simulink model "model"  (R2016a)
(part 9 of 10)

  _CN_101346507_220000_CN_101346508_220000/RConn1 -- T_101346508_220000_Ital_Novi/LConn1 -- Vignole_Ilva_CN_101346508_220000_CN_100952845_220000/RConn1
  _CN_101346507_220000_CN_101346508_220000/RConn2 -- T_101346508_220000_Ital_Novi/LConn2 -- Vignole_Ilva_CN_101346508_220000_CN_100952845_220000/RConn2
  _CN_101346507_220000_CN_101346508_220000/RConn3 -- T_101346508_220000_Ital_Novi/LConn3 -- Vignole_Ilva_CN_101346508_220000_CN_100952845_220000/RConn3 -- bus206/LConn1
  T_95466193_220000_/LConn1 -- Roma_Sud_Cinecittà_CN_95466193_220000_CN_76705565_220000/LConn1
  T_95466193_220000_/LConn2 -- Roma_Sud_Cinecittà_CN_95466193_220000_CN_76705565_220000/LConn2
  Roma_Sud_Cinecittà_CN_95466193_220000_CN_76705565_220000/LConn3 -- T_95466193_220000_/LConn3 -- bus207/LConn1
  Roma_Sud_Cinecittà_CN_95466193_220000_CN_76705565_220000/RConn1 -- T_76705565_380000;220000;150000_Roma_Sud/RConn1 -- Roma_Sud_San_Paolo_CN_76705565_220000_CN_95466377_220000/LConn1
  Roma_Sud_Cinecittà_CN_95466193_220000_CN_76705565_220000/RConn2 -- T_76705565_380000;220000;150000_Roma_Sud/RConn2 -- Roma_Sud_San_Paolo_CN_76705565_220000_CN_95466377_220000/LConn2
  Roma_Sud_Cinecittà_CN_95466193_220000_CN_76705565_220000/RConn3 -- T_76705565_380000;220000;150000_Roma_Sud/RConn3 -- Roma_Sud_San_Paolo_CN_76705565_220000_CN_95466377_220000/LConn3 -- bus208/LConn1
  _CN_375916035_220000_CN_56984450_220000/RConn1 -- T_375916035_220000_Cattolica_Eraclea_centrale/LConn1 -- _CN_375916035_220000_CN_53635045_220000/RConn1 -- _CN_375916035_220000_CN_375907988_220000/LConn1
  _CN_375916035_220000_CN_56984450_220000/RConn2 -- T_375916035_220000_Cattolica_Eraclea_centrale/LConn2 -- _CN_375916035_220000_CN_53635045_220000/RConn2 -- _CN_375916035_220000_CN_375907988_220000/LConn2
  _CN_375916035_220000_CN_56984450_220000/RConn3 -- T_375916035_220000_Cattolica_Eraclea_centrale/LConn3 -- _CN_375916035_220000_CN_53635045_220000/RConn3 -- _CN_375916035_220000_CN_375907988_220000/LConn3 -- bus209/LConn1
  T_375907988_220000_Sambuca/LConn1 -- _CN_375916035_220000_CN_375907988_220000/RConn1
  T_375907988_220000_Sambuca/LConn2 -- _CN_375916035_220000_CN_375907988_220000/RConn2
  _CN_375916035_220000_CN_375907988_220000/RConn3 -- T_375907988_220000_Sambuca/LConn3 -- bus210/LConn1
  Patria_Pozzuoli_CN_114661587_220000_CN_132726160_220000/RConn1 -- T_132726160_220000_Pozzuoli/LConn1 -- Astroni_Pozzuoli_CN_132726160_220000_CN_132725149_220000/RConn1
  Patria_Pozzuoli_CN_114661587_220000_CN_132726160_220000/RConn2 -- T_132726160_220000_Pozzuoli/LConn2 -- Astroni_Pozzuoli_CN_132726160_220000_CN_132725149_220000/RConn2
  Patria_Pozzuoli_CN_114661587_220000_CN_132726160_220000/RConn3 -- T_132726160_220000_Pozzuoli/LConn3 -- Astroni_Pozzuoli_CN_132726160_220000_CN_132725149_220000/RConn3 -- bus211/LConn1
  T_377832777_220000_Tirano/LConn1 -- Cesano_Maderno_Tirano_CN_74359510_220000_CN_377832777_220000/RConn1
  T_377832777_220000_Tirano/LConn2 -- Cesano_Maderno_Tirano_CN_74359510_220000_CN_377832777_220000/RConn2
  Cesano_Maderno_Tirano_CN_74359510_220000_CN_377832777_220000/RConn3 -- T_377832777_220000_Tirano/LConn3 -- bus212/LConn1
  Cesano_Maderno_Tirano_CN_74359510_220000_CN_98787157_220000/RConn1 -- T_98787157_220000_Glorenza/LConn1 -- _CN_98787157_220000_CN96653153/LConn1
  Cesano_Maderno_Tirano_CN_74359510_220000_CN_98787157_220000/RConn2 -- T_98787157_220000_Glorenza/LConn2 -- _CN_98787157_220000_CN96653153/LConn2
  Cesano_Maderno_Tirano_CN_74359510_220000_CN_98787157_220000/RConn3 -- T_98787157_220000_Glorenza/LConn3 -- _CN_98787157_220000_CN96653153/LConn3 -- bus213/LConn1
  T_377588184_220000_Caivano/LConn1 -- Fratta_Maddaloni_CN_132702940_220000_CN_377588184_220000/RConn1
  T_377588184_220000_Caivano/LConn2 -- Fratta_Maddaloni_CN_132702940_220000_CN_377588184_220000/RConn2
  Fratta_Maddaloni_CN_132702940_220000_CN_377588184_220000/RConn3 -- T_377588184_220000_Caivano/LConn3 -- bus214/LConn1
  T_132719324_220000_Air_Liquide/LConn1 -- Maddaloni_Air_Liquide_CN_132719324_220000_CN_132717802_220000/RConn1
  T_132719324_220000_Air_Liquide/LConn2 -- Maddaloni_Air_Liquide_CN_132719324_220000_CN_132717802_220000/RConn2
  Maddaloni_Air_Liquide_CN_132719324_220000_CN_132717802_220000/RConn3 -- T_132719324_220000_Air_Liquide/LConn3 -- bus215/LConn1
  T_84696559_380000_Santa_Sofia/RConn4 -- Maddaloni_Santa_Sofia_CN_132717802_220000_CN_84696559_220000/RConn1
  T_84696559_380000_Santa_Sofia/RConn5 -- Maddaloni_Santa_Sofia_CN_132717802_220000_CN_84696559_220000/RConn2
  Maddaloni_Santa_Sofia_CN_132717802_220000_CN_84696559_220000/RConn3 -- T_84696559_380000_Santa_Sofia/RConn6 -- bus216/LConn1
  T_162960205_380000_Tavazzano_Centrale/RConn4 -- _CN_116916459_220000_CN_162960205_220000/RConn1
  T_162960205_380000_Tavazzano_Centrale/RConn5 -- _CN_116916459_220000_CN_162960205_220000/RConn2
  _CN_116916459_220000_CN_162960205_220000/RConn3 -- T_162960205_380000_Tavazzano_Centrale/RConn6 -- bus217/LConn1
  T_214294769_220000_Moline/LConn1 -- _CN_214294769_220000_CN_103549584_220000/RConn1
  T_214294769_220000_Moline/LConn2 -- _CN_214294769_220000_CN_103549584_220000/RConn2
  _CN_214294769_220000_CN_103549584_220000/RConn3 -- T_214294769_220000_Moline/LConn3 -- bus218/LConn1
  T_281837810_220000_Cedegolo_Sud/LConn1 -- Taio_Cedegolo_CN_281837810_220000_CN96654904/RConn1
  T_281837810_220000_Cedegolo_Sud/LConn2 -- Taio_Cedegolo_CN_281837810_220000_CN96654904/RConn2
  Taio_Cedegolo_CN_281837810_220000_CN96654904/RConn3 -- T_281837810_220000_Cedegolo_Sud/LConn3 -- bus219/LConn1
  T_181125039_220000_Enipower_Ferrara/LConn1 -- Bussolengo_Ferrara_CN_111020792_220000_CN_181125039_220000/RConn1
  T_181125039_220000_Enipower_Ferrara/LConn2 -- Bussolengo_Ferrara_CN_111020792_220000_CN_181125039_220000/RConn2
  Bussolengo_Ferrara_CN_111020792_220000_CN_181125039_220000/RConn3 -- T_181125039_220000_Enipower_Ferrara/LConn3 -- bus220/LConn1
  T_82078641_380000_Ostiglia/RConn4 -- Mincio_Colunga_CN_111020792_220000_CN_82078641_220000/RConn1
  T_82078641_380000_Ostiglia/RConn5 -- Mincio_Colunga_CN_111020792_220000_CN_82078641_220000/RConn2
  Mincio_Colunga_CN_111020792_220000_CN_82078641_220000/RConn3 -- T_82078641_380000_Ostiglia/RConn6 -- bus221/LConn1
  T_162066058_220000_Verona_Borgomilano/LConn1 -- _CN_111020792_220000_CN_162066058_220000/RConn1
  T_162066058_220000_Verona_Borgomilano/LConn2 -- _CN_111020792_220000_CN_162066058_220000/RConn2
  _CN_111020792_220000_CN_162066058_220000/RConn3 -- T_162066058_220000_Verona_Borgomilano/LConn3 -- bus222/LConn1
  T_289178949_220000_Riva_Acciaio/LConn1 -- _CN_111020792_220000_CN_289178949_220000/RConn1
  T_289178949_220000_Riva_Acciaio/LConn2 -- _CN_111020792_220000_CN_289178949_220000/RConn2
  _CN_111020792_220000_CN_289178949_220000/RConn3 -- T_289178949_220000_Riva_Acciaio/LConn3 -- bus223/LConn1
  T_103725446_220000_Sondel_Settimo_Torinese/LConn1 -- Stura_Sondel_CN_103725268_220000_CN_103725446_220000/RConn1
  T_103725446_220000_Sondel_Settimo_Torinese/LConn2 -- Stura_Sondel_CN_103725268_220000_CN_103725446_220000/RConn2
  Stura_Sondel_CN_103725268_220000_CN_103725446_220000/RConn3 -- T_103725446_220000_Sondel_Settimo_Torinese/LConn3 -- bus224/LConn1
  T_82767145_380000_Tirreno_Power_Torrevaldaliga/RConn4 -- Torrevaldaliga_Sud_Santa_Lucia_CN_82762493_220000_CN_82767145_220000/RConn1
  T_82767145_380000_Tirreno_Power_Torrevaldaliga/RConn5 -- Torrevaldaliga_Sud_Santa_Lucia_CN_82762493_220000_CN_82767145_220000/RConn2
  Torrevaldaliga_Sud_Santa_Lucia_CN_82762493_220000_CN_82767145_220000/RConn3 -- T_82767145_380000_Tirreno_Power_Torrevaldaliga/RConn6 -- bus225/LConn1
  T_194186027_220000_Duferdofin/LConn1 -- Sorgente___Duferdofin_CN_194186027_220000_CN_110138220_220000/RConn1
  T_194186027_220000_Duferdofin/LConn2 -- Sorgente___Duferdofin_CN_194186027_220000_CN_110138220_220000/RConn2
  Sorgente___Duferdofin_CN_194186027_220000_CN_110138220_220000/RConn3 -- T_194186027_220000_Duferdofin/LConn3 -- bus226/LConn1
  T_338948868_220000_Termini_Centrale_gruppi_6/LConn1 -- _CN_338948868_220000_CN53456167/LConn1
  T_338948868_220000_Termini_Centrale_gruppi_6/LConn2 -- _CN_338948868_220000_CN53456167/LConn2
  _CN_338948868_220000_CN53456167/LConn3 -- T_338948868_220000_Termini_Centrale_gruppi_6/LConn3 -- bus227/LConn1
  _CN_338948868_220000_CN53456167/RConn1 -- "G_53456167_Centrale_termoelettrica_\"Ettore_Maiorana\""/RConn1 -- _CN_57736553_220000_CN53456167/RConn1
  _CN_338948868_220000_CN53456167/RConn2 -- "G_53456167_Centrale_termoelettrica_\"Ettore_Maiorana\""/RConn2 -- _CN_57736553_220000_CN53456167/RConn2
  _CN_338948868_220000_CN53456167/RConn3 -- "G_53456167_Centrale_termoelettrica_\"Ettore_Maiorana\""/RConn3 -- _CN_57736553_220000_CN53456167/RConn3 -- bus228/LConn1
  T_145665797_220000_Brindisi_Nord_220/LConn1 -- Brindisi_Brindisi_Nord_CN_145665797_220000_CN402304796/LConn1
  T_145665797_220000_Brindisi_Nord_220/LConn2 -- Brindisi_Brindisi_Nord_CN_145665797_220000_CN402304796/LConn2
  Brindisi_Brindisi_Nord_CN_145665797_220000_CN402304796/LConn3 -- T_145665797_220000_Brindisi_Nord_220/LConn3 -- bus229/LConn1
  Brindisi_Brindisi_Nord_CN_145665797_220000_CN402304796/RConn1 -- G_402304796_Centrale_termoelettrica_di_Brindisi/RConn1 -- Brindisi_Brindisi_Nord_CN_60919237_220000_CN402304796/LConn1
  Brindisi_Brindisi_Nord_CN_145665797_220000_CN402304796/RConn2 -- G_402304796_Centrale_termoelettrica_di_Brindisi/RConn2 -- Brindisi_Brindisi_Nord_CN_60919237_220000_CN402304796/LConn2
  Brindisi_Brindisi_Nord_CN_145665797_220000_CN402304796/RConn3 -- G_402304796_Centrale_termoelettrica_di_Brindisi/RConn3 -- Brindisi_Brindisi_Nord_CN_60919237_220000_CN402304796/LConn3 -- bus230/LConn1
  T_103653591_220000_Vado_Stazione/LConn1 -- Savona_Vado_Ligure_CN_103653591_220000_CN_296141722_220000/RConn1
  T_103653591_220000_Vado_Stazione/LConn2 -- Savona_Vado_Ligure_CN_103653591_220000_CN_296141722_220000/RConn2
  Savona_Vado_Ligure_CN_103653591_220000_CN_296141722_220000/RConn3 -- T_103653591_220000_Vado_Stazione/LConn3 -- bus231/LConn1
  T_100407576_380000_Fusina_Termica_sezione_1_220/RConn1 -- Dolo___Fusina_CN_100407576_220000_CN_59153311_220000/RConn1
  T_100407576_380000_Fusina_Termica_sezione_1_220/RConn2 -- Dolo___Fusina_CN_100407576_220000_CN_59153311_220000/RConn2
  Dolo___Fusina_CN_100407576_220000_CN_59153311_220000/RConn3 -- T_100407576_380000_Fusina_Termica_sezione_1_220/RConn3 -- bus232/LConn1
  T_95466377_220000_/LConn1 -- Roma_Sud_San_Paolo_CN_76705565_220000_CN_95466377_220000/RConn1
  T_95466377_220000_/LConn2 -- Roma_Sud_San_Paolo_CN_76705565_220000_CN_95466377_220000/RConn2
  Roma_Sud_San_Paolo_CN_76705565_220000_CN_95466377_220000/RConn3 -- T_95466377_220000_/LConn3 -- bus233/LConn1
  Villa___Rosone_CN_66872608_220000_CN_102185356_220000/RConn1 -- T_102185356_220000_Villa/LConn1 -- Villeneuve_Villa_CN_102185356_220000_CN_102185362_220000/RConn1
  Villa___Rosone_CN_66872608_220000_CN_102185356_220000/RConn2 -- T_102185356_220000_Villa/LConn2 -- Villeneuve_Villa_CN_102185356_220000_CN_102185362_220000/RConn2
  Villa___Rosone_CN_66872608_220000_CN_102185356_220000/RConn3 -- T_102185356_220000_Villa/LConn3 -- Villeneuve_Villa_CN_102185356_220000_CN_102185362_220000/RConn3 -- bus234/LConn1
  T_162828577_380000_Turbigo/RConn4 -- Biella_Est___Turbigo_CN_162828577_220000_CN_82651599_220000/RConn1
  T_162828577_380000_Turbigo/RConn5 -- Biella_Est___Turbigo_CN_162828577_220000_CN_82651599_220000/RConn2
  Biella_Est___Turbigo_CN_162828577_220000_CN_82651599_220000/RConn3 -- T_162828577_380000_Turbigo/RConn6 -- bus235/LConn1
  T_136708548_220000_Certosa/LConn1 -- _CN_62326314_220000_CN_136708548_220000/RConn1
  T_136708548_220000_Certosa/LConn2 -- _CN_62326314_220000_CN_136708548_220000/RConn2
  _CN_62326314_220000_CN_136708548_220000/RConn3 -- T_136708548_220000_Certosa/LConn3 -- bus236/LConn1
  T_118987056_380000_Selargius/RConn4 -- Selargius_Villasor_CN_118987056_220000_CN_144005861_220000/RConn1
  T_118987056_380000_Selargius/RConn5 -- Selargius_Villasor_CN_118987056_220000_CN_144005861_220000/RConn2
  Selargius_Villasor_CN_118987056_220000_CN_144005861_220000/RConn3 -- T_118987056_380000_Selargius/RConn6 -- bus237/LConn1
  Colli_Aminei_Secondigliano_CN_377444657_220000_CN_376502663_220000/RConn1 -- T_377444657_220000_Secondigliano/LConn1 -- Fratta_Secondigliano_CN_377444657_220000_CN_377444648_220000/RConn1
  Colli_Aminei_Secondigliano_CN_377444657_220000_CN_376502663_220000/RConn2 -- T_377444657_220000_Secondigliano/LConn2 -- Fratta_Secondigliano_CN_377444657_220000_CN_377444648_220000/RConn2
  Colli_Aminei_Secondigliano_CN_377444657_220000_CN_376502663_220000/RConn3 -- T_377444657_220000_Secondigliano/LConn3 -- Fratta_Secondigliano_CN_377444657_220000_CN_377444648_220000/RConn3 -- bus238/LConn1
  _CN_172705586_220000_CN_57736541_220000/LConn1 -- T_172705586__Bellolampo/LConn1 -- _CN_172705586_220000_CN_57736553_220000/RConn1
  _CN_172705586_220000_CN_57736541_220000/LConn2 -- T_172705586__Bellolampo/LConn2 -- _CN_172705586_220000_CN_57736553_220000/RConn2
  _CN_172705586_220000_CN_57736541_220000/LConn3 -- T_172705586__Bellolampo/LConn3 -- _CN_172705586_220000_CN_57736553_220000/RConn3 -- bus239/LConn1
  _CN_172705586_220000_CN_57736541_220000/RConn1 -- T_57736541__Partinico/LConn1 -- _CN_57736541_220000_CN_57403755_220000/LConn1 -- _CN_57736541_220000_CN_53635045_220000/RConn1
  _CN_172705586_220000_CN_57736541_220000/RConn2 -- T_57736541__Partinico/LConn2 -- _CN_57736541_220000_CN_57403755_220000/LConn2 -- _CN_57736541_220000_CN_53635045_220000/RConn2
  _CN_172705586_220000_CN_57736541_220000/RConn3 -- T_57736541__Partinico/LConn3 -- _CN_57736541_220000_CN_57403755_220000/LConn3 -- _CN_57736541_220000_CN_53635045_220000/RConn3 -- bus240/LConn1
  _CN_103007030_220000_CN_103007085_220000/LConn1 -- T_103007030_220000_Chatillon_Centrale/LConn1 -- _CN_103007030_220000_CN_103127417_220000/LConn1 -- _CN_103007030_220000_CN_102185362_220000/RConn1 -- _CN_103007030_220000_CN_105153431_220000/LConn1
  _CN_103007030_220000_CN_103007085_220000/LConn2 -- T_103007030_220000_Chatillon_Centrale/LConn2 -- _CN_103007030_220000_CN_103127417_220000/LConn2 -- _CN_103007030_220000_CN_102185362_220000/RConn2 -- _CN_103007030_220000_CN_105153431_220000/LConn2
  _CN_103007030_220000_CN_103007085_220000/LConn3 -- T_103007030_220000_Chatillon_Centrale/LConn3 -- _CN_103007030_220000_CN_103127417_220000/LConn3 -- _CN_103007030_220000_CN_102185362_220000/RConn3 -- bus241/LConn1 -- _CN_103007030_220000_CN_105153431_220000/LConn3
  T_103007085_220000_Montjovet_centrale/LConn1 -- _CN_103007030_220000_CN_103007085_220000/RConn1
  T_103007085_220000_Montjovet_centrale/LConn2 -- _CN_103007030_220000_CN_103007085_220000/RConn2
  _CN_103007030_220000_CN_103007085_220000/RConn3 -- T_103007085_220000_Montjovet_centrale/LConn3 -- bus242/LConn1
  _CN_103007030_220000_CN_105153431_220000/RConn1 -- T_105153431_380000_Leinì/RConn4 -- _CN_74869121_220000_CN_105153431_220000/RConn1 -- _CN_105153431_220000_CN_332123606_220000/RConn1
  _CN_103007030_220000_CN_105153431_220000/RConn2 -- T_105153431_380000_Leinì/RConn5 -- _CN_74869121_220000_CN_105153431_220000/RConn2 -- _CN_105153431_220000_CN_332123606_220000/RConn2
  _CN_103007030_220000_CN_105153431_220000/RConn3 -- T_105153431_380000_Leinì/RConn6 -- _CN_74869121_220000_CN_105153431_220000/RConn3 -- _CN_105153431_220000_CN_332123606_220000/RConn3 -- bus243/LConn1
  T_103127417_220000_Valpelline_G2/LConn1 -- _CN_103007030_220000_CN_103127417_220000/RConn1
  T_103127417_220000_Valpelline_G2/LConn2 -- _CN_103007030_220000_CN_103127417_220000/RConn2
  _CN_103007030_220000_CN_103127417_220000/RConn3 -- T_103127417_220000_Valpelline_G2/LConn3 -- bus244/LConn1
  T_189137043_220000_Gargnano/LConn1 -- Gargnano_Nave_CN_189137043_220000_CN_147466201_220000/RConn1
  T_189137043_220000_Gargnano/LConn2 -- Gargnano_Nave_CN_189137043_220000_CN_147466201_220000/RConn2
  Gargnano_Nave_CN_189137043_220000_CN_147466201_220000/RConn3 -- T_189137043_220000_Gargnano/LConn3 -- bus245/LConn1
  G_139974542_Centrale_elettrica_Taloro/RConn1 -- Ottana_Taloro_1_CN_144006711_220000_CN139974542/RConn1
  G_139974542_Centrale_elettrica_Taloro/RConn2 -- Ottana_Taloro_1_CN_144006711_220000_CN139974542/RConn2
  Ottana_Taloro_1_CN_144006711_220000_CN139974542/RConn3 -- G_139974542_Centrale_elettrica_Taloro/RConn3 -- bus246/LConn1
  T_320030656_220000_Tecnoparco/LConn1 -- Pisticci_Tecnoparco_CN_104321356_220000_CN_320030656_220000/RConn1
  T_320030656_220000_Tecnoparco/LConn2 -- Pisticci_Tecnoparco_CN_104321356_220000_CN_320030656_220000/RConn2
  Pisticci_Tecnoparco_CN_104321356_220000_CN_320030656_220000/RConn3 -- T_320030656_220000_Tecnoparco/LConn3 -- bus247/LConn1
  T_348500306_220000_Campo_Moro/LConn1 -- Lanzada_Campo_Moro_CN_348500306_220000_CN_163056526_220000/RConn1
  T_348500306_220000_Campo_Moro/LConn2 -- Lanzada_Campo_Moro_CN_348500306_220000_CN_163056526_220000/RConn2
  Lanzada_Campo_Moro_CN_348500306_220000_CN_163056526_220000/RConn3 -- T_348500306_220000_Campo_Moro/LConn3 -- bus248/LConn1
  G_96653153_Kraftwerk_Kastelbell___Centrale_idroelettrica_di_Castelbello/RConn1 -- _CN_98787157_220000_CN96653153/RConn1
  G_96653153_Kraftwerk_Kastelbell___Centrale_idroelettrica_di_Castelbello/RConn2 -- _CN_98787157_220000_CN96653153/RConn2
  _CN_98787157_220000_CN96653153/RConn3 -- G_96653153_Kraftwerk_Kastelbell___Centrale_idroelettrica_di_Castelbello/RConn3 -- bus249/LConn1
  T_105581403_380000_Chivasso_Termica_380kV/RConn4 -- _CN_105581403_220000_CN_102287716_220000/LConn1
  T_105581403_380000_Chivasso_Termica_380kV/RConn5 -- _CN_105581403_220000_CN_102287716_220000/LConn2
  _CN_105581403_220000_CN_102287716_220000/LConn3 -- T_105581403_380000_Chivasso_Termica_380kV/RConn6 -- bus250/LConn1
  _CN_105581403_220000_CN_102287716_220000/RConn1 -- T_102287716_220000_Chivasso_Termica_220kV/LConn1 -- Chivasso_Termica___Rondissone_CN_102287716_220000_CN_74869121_220000/RConn1 -- _CN_102287716_220000_CN95099552/LConn1
  _CN_105581403_220000_CN_102287716_220000/RConn2 -- T_102287716_220000_Chivasso_Termica_220kV/LConn2 -- Chivasso_Termica___Rondissone_CN_102287716_220000_CN_74869121_220000/RConn2 -- _CN_102287716_220000_CN95099552/LConn2
  _CN_105581403_220000_CN_102287716_220000/RConn3 -- T_102287716_220000_Chivasso_Termica_220kV/LConn3 -- Chivasso_Termica___Rondissone_CN_102287716_220000_CN_74869121_220000/RConn3 -- _CN_102287716_220000_CN95099552/LConn3 -- bus251/LConn1
  _CN_57736541_220000_CN_57403755_220000/RConn1 -- T_57403755_220000_Ciminna/LConn1 -- _CN_57736553_220000_CN_57403755_220000/RConn1
  _CN_57736541_220000_CN_57403755_220000/RConn2 -- T_57403755_220000_Ciminna/LConn2 -- _CN_57736553_220000_CN_57403755_220000/RConn2
  _CN_57736541_220000_CN_57403755_220000/RConn3 -- T_57403755_220000_Ciminna/LConn3 -- _CN_57736553_220000_CN_57403755_220000/RConn3 -- bus252/LConn1
  T_207383904_220000_Arenella/LConn1 -- _CN_207383904_220000_CN_377588144_220000/LConn1
  T_207383904_220000_Arenella/LConn2 -- _CN_207383904_220000_CN_377588144_220000/LConn2
  _CN_207383904_220000_CN_377588144_220000/LConn3 -- T_207383904_220000_Arenella/LConn3 -- bus253/LConn1
  _CN_207383904_220000_CN_377588144_220000/RConn1 -- T_377588144_220000_/LConn1 -- Astroni_Arenella_CN_132725149_220000_CN_377588144_220000/RConn1 -- Colli_Aminei_Arenella_CN_376502663_220000_CN_377588144_220000/RConn1
  _CN_207383904_220000_CN_377588144_220000/RConn2 -- T_377588144_220000_/LConn2 -- Astroni_Arenella_CN_132725149_220000_CN_377588144_220000/RConn2 -- Colli_Aminei_Arenella_CN_376502663_220000_CN_377588144_220000/RConn2
  _CN_207383904_220000_CN_377588144_220000/RConn3 -- T_377588144_220000_/LConn3 -- Astroni_Arenella_CN_132725149_220000_CN_377588144_220000/RConn3 -- Colli_Aminei_Arenella_CN_376502663_220000_CN_377588144_220000/RConn3 -- bus254/LConn1
  T_149071351_220000_Acciaieria_Valsugana/LConn1 -- Borgo_Valsugana_Acciaieria_CN_103549584_220000_CN_149071351_220000/RConn1
  T_149071351_220000_Acciaieria_Valsugana/LConn2 -- Borgo_Valsugana_Acciaieria_CN_103549584_220000_CN_149071351_220000/RConn2
  Borgo_Valsugana_Acciaieria_CN_103549584_220000_CN_149071351_220000/RConn3 -- T_149071351_220000_Acciaieria_Valsugana/LConn3 -- bus255/LConn1
  G_95099552_Centrale_Termoelettrica_di_Chivasso/RConn1 -- _CN_102287716_220000_CN95099552/RConn1
  G_95099552_Centrale_Termoelettrica_di_Chivasso/RConn2 -- _CN_102287716_220000_CN95099552/RConn2
  _CN_102287716_220000_CN95099552/RConn3 -- G_95099552_Centrale_Termoelettrica_di_Chivasso/RConn3 -- bus256/LConn1
  T_147453809_220000_Santa_Massenza_sezione_220K/LConn1 -- _CN_147453809_220000_CN_147466201_220000/RConn1
  T_147453809_220000_Santa_Massenza_sezione_220K/LConn2 -- _CN_147453809_220000_CN_147466201_220000/RConn2
  _CN_147453809_220000_CN_147466201_220000/RConn3 -- T_147453809_220000_Santa_Massenza_sezione_220K/LConn3 -- bus257/LConn1
  T_107683818_380000_Stazione_elettrica_Marginone/RConn4 -- Marginone__Livorno_Marzocco_CN_107683818_220000_CN_107843509_220000/LConn1
  T_107683818_380000_Stazione_elettrica_Marginone/RConn5 -- Marginone__Livorno_Marzocco_CN_107683818_220000_CN_107843509_220000/LConn2
  Marginone__Livorno_Marzocco_CN_107683818_220000_CN_107843509_220000/LConn3 -- T_107683818_380000_Stazione_elettrica_Marginone/RConn6 -- bus258/LConn1
  T_107843509_220000_Livorno_Marzocco/LConn1 -- Marginone__Livorno_Marzocco_CN_107683818_220000_CN_107843509_220000/RConn1
  T_107843509_220000_Livorno_Marzocco/LConn2 -- Marginone__Livorno_Marzocco_CN_107683818_220000_CN_107843509_220000/RConn2
  Marginone__Livorno_Marzocco_CN_107683818_220000_CN_107843509_220000/RConn3 -- T_107843509_220000_Livorno_Marzocco/LConn3 -- bus259/LConn1
  T_375922075_220000_Eni_Versalis/LConn1 -- Ragusa_Polimeri_Europa_CN_375922075_220000_CN_57380344_220000/RConn1
  T_375922075_220000_Eni_Versalis/LConn2 -- Ragusa_Polimeri_Europa_CN_375922075_220000_CN_57380344_220000/RConn2
  Ragusa_Polimeri_Europa_CN_375922075_220000_CN_57380344_220000/RConn3 -- T_375922075_220000_Eni_Versalis/LConn3 -- bus260/LConn1
  Villa_Castelli_Brindisi_CN_377300897_220000_CN_60919237_220000/RConn1 -- T_60919237_380000_Brindisi/RConn4 -- Brindisi_Brindisi_Nord_CN_60919237_220000_CN402304796/RConn1
  Villa_Castelli_Brindisi_CN_377300897_220000_CN_60919237_220000/RConn2 -- T_60919237_380000_Brindisi/RConn5 -- Brindisi_Brindisi_Nord_CN_60919237_220000_CN402304796/RConn2
  Villa_Castelli_Brindisi_CN_377300897_220000_CN_60919237_220000/RConn3 -- T_60919237_380000_Brindisi/RConn6 -- Brindisi_Brindisi_Nord_CN_60919237_220000_CN402304796/RConn3 -- bus261/LConn1
  T_377438327_220000_Imi_sud/LConn1 -- Casoria_Imi_sud_CN_377438327_220000_CN_376502734_220000/RConn1
  T_377438327_220000_Imi_sud/LConn2 -- Casoria_Imi_sud_CN_377438327_220000_CN_376502734_220000/RConn2
  Casoria_Imi_sud_CN_377438327_220000_CN_376502734_220000/RConn3 -- T_377438327_220000_Imi_sud/LConn3 -- bus262/LConn1
  T_82793962_220000_Cimego/LConn1 -- Cimego_Santa_Massenza_CN_147466201_220000_CN_82793962_220000/RConn1
  T_82793962_220000_Cimego/LConn2 -- Cimego_Santa_Massenza_CN_147466201_220000_CN_82793962_220000/RConn2
  Cimego_Santa_Massenza_CN_147466201_220000_CN_82793962_220000/RConn3 -- T_82793962_220000_Cimego/LConn3 -- bus263/LConn1
  _CN_339706880_380000_CN_59219335_380000/LConn1 -- T_339706880_380000_Tuscania/LConn1 -- _CN_339706880_380000_CN_61375111_380000/LConn1 -- _CN_339706880_380000_CN_339706881_380000/LConn1
  _CN_339706880_380000_CN_59219335_380000/LConn2 -- T_339706880_380000_Tuscania/LConn2 -- _CN_339706880_380000_CN_61375111_380000/LConn2 -- _CN_339706880_380000_CN_339706881_380000/LConn2
  _CN_339706880_380000_CN_59219335_380000/LConn3 -- T_339706880_380000_Tuscania/LConn3 -- _CN_339706880_380000_CN_61375111_380000/LConn3 -- _CN_339706880_380000_CN_339706881_380000/LConn3 -- bus264/LConn1
  _CN_339706880_380000_CN_59219335_380000/RConn1 -- T_59219335_380000_Montalto/LConn1 -- _CN_59219335_380000_CN96951146/LConn1 -- _CN_59219335_380000_CN161471016/LConn1 -- Pian_della_Speranza___Roma_Nord_CN_83805453_380000_CN_59219335_380000/LConn1 -- _CN_82759380_380000_CN_59219335_380000/LConn1
  _CN_339706880_380000_CN_59219335_380000/RConn2 -- T_59219335_380000_Montalto/LConn2 -- _CN_59219335_380000_CN96951146/LConn2 -- _CN_59219335_380000_CN161471016/LConn2 -- Pian_della_Speranza___Roma_Nord_CN_83805453_380000_CN_59219335_380000/LConn2 -- _CN_82759380_380000_CN_59219335_380000/LConn2
  _CN_339706880_380000_CN_59219335_380000/RConn3 -- T_59219335_380000_Montalto/LConn3 -- _CN_59219335_380000_CN96951146/LConn3 -- _CN_59219335_380000_CN161471016/LConn3 -- bus265/LConn1 -- Pian_della_Speranza___Roma_Nord_CN_83805453_380000_CN_59219335_380000/LConn3 -- _CN_82759380_380000_CN_59219335_380000/LConn3
  _CN_339706880_380000_CN_61375111_380000/RConn1 -- T_61375111_380000_Villanova/LConn1 -- Teramo_Villanova_CN_61375111_380000_CN_61626687_380000/LConn1 -- _CN_61375111_380000_CN_60616350_380000/LConn1
  _CN_339706880_380000_CN_61375111_380000/RConn2 -- T_61375111_380000_Villanova/LConn2 -- Teramo_Villanova_CN_61375111_380000_CN_61626687_380000/LConn2 -- _CN_61375111_380000_CN_60616350_380000/LConn2
  _CN_339706880_380000_CN_61375111_380000/RConn3 -- T_61375111_380000_Villanova/LConn3 -- Teramo_Villanova_CN_61375111_380000_CN_61626687_380000/LConn3 -- _CN_61375111_380000_CN_60616350_380000/LConn3 -- bus266/LConn1
  T_339706881_380000_Villavalle/LConn1 -- _CN_339706880_380000_CN_339706881_380000/RConn1
  T_339706881_380000_Villavalle/LConn2 -- _CN_339706880_380000_CN_339706881_380000/RConn2
  _CN_339706880_380000_CN_339706881_380000/RConn3 -- T_339706881_380000_Villavalle/LConn3 -- bus267/LConn1
  Bari_ovest_Brindisi_CN_60913666_380000_CN_60919237_380000/LConn1 -- T_60913666_380000_Bari_Ovest/LConn1 -- Bari_Ovest_Palo_del_Colle_CN_60913666_380000_CN_146791061_380000/LConn1
  Bari_ovest_Brindisi_CN_60913666_380000_CN_60919237_380000/LConn2 -- T_60913666_380000_Bari_Ovest/LConn2 -- Bari_Ovest_Palo_del_Colle_CN_60913666_380000_CN_146791061_380000/LConn2
  Bari_ovest_Brindisi_CN_60913666_380000_CN_60919237_380000/LConn3 -- T_60913666_380000_Bari_Ovest/LConn3 -- Bari_Ovest_Palo_del_Colle_CN_60913666_380000_CN_146791061_380000/LConn3 -- bus268/LConn1
  Bari_ovest_Brindisi_CN_60913666_380000_CN_60919237_380000/RConn1 -- T_60919237_380000_Brindisi/LConn1 -- _CN_145665799_380000_CN_60919237_380000/LConn1 -- _CN_60888331_380000_CN_60919237_380000/LConn1 -- _CN_145665323_380000_CN_60919237_380000/LConn1 -- Brindisi_Taranto_nord_CN_103381531_380000_CN_60919237_380000/LConn1
  Bari_ovest_Brindisi_CN_60913666_380000_CN_60919237_380000/RConn2 -- T_60919237_380000_Brindisi/LConn2 -- _CN_145665799_380000_CN_60919237_380000/LConn2 -- _CN_60888331_380000_CN_60919237_380000/LConn2 -- _CN_145665323_380000_CN_60919237_380000/LConn2 -- Brindisi_Taranto_nord_CN_103381531_380000_CN_60919237_380000/LConn2
  Bari_ovest_Brindisi_CN_60913666_380000_CN_60919237_380000/RConn3 -- T_60919237_380000_Brindisi/LConn3 -- _CN_145665799_380000_CN_60919237_380000/LConn3 -- _CN_60888331_380000_CN_60919237_380000/LConn3 -- _CN_145665323_380000_CN_60919237_380000/LConn3 -- bus269/LConn1 -- Brindisi_Taranto_nord_CN_103381531_380000_CN_60919237_380000/LConn3
  Bari_Ovest_Palo_del_Colle_CN_60913666_380000_CN_146791061_380000/RConn1 -- T_146791061_380000_Palo_del_Colle/LConn1 -- Foggia_Palo_del_Colle_CN_418565263_380000_CN_146791061_380000/LConn1 -- _CN_146791061_380000_CN_146791215_380000/LConn1
  Bari_Ovest_Palo_del_Colle_CN_60913666_380000_CN_146791061_380000/RConn2 -- T_146791061_380000_Palo_del_Colle/LConn2 -- Foggia_Palo_del_Colle_CN_418565263_380000_CN_146791061_380000/LConn2 -- _CN_146791061_380000_CN_146791215_380000/LConn2
  Bari_Ovest_Palo_del_Colle_CN_60913666_380000_CN_146791061_380000/RConn3 -- T_146791061_380000_Palo_del_Colle/LConn3 -- Foggia_Palo_del_Colle_CN_418565263_380000_CN_146791061_380000/LConn3 -- _CN_146791061_380000_CN_146791215_380000/LConn3 -- bus270/LConn1
  T_416989699_380000_Montalto_centrale/LConn1 -- _CN_416989699_380000_CN96951146/LConn1
  T_416989699_380000_Montalto_centrale/LConn2 -- _CN_416989699_380000_CN96951146/LConn2
  _CN_416989699_380000_CN96951146/LConn3 -- T_416989699_380000_Montalto_centrale/LConn3 -- bus271/LConn1
  _CN_416989699_380000_CN96951146/RConn1 -- "G_96951146_Centrale_termoelettrica_\"Alessandro_Volta\""/RConn1 -- _CN_59219335_380000_CN96951146/RConn1
  _CN_416989699_380000_CN96951146/RConn2 -- "G_96951146_Centrale_termoelettrica_\"Alessandro_Volta\""/RConn2 -- _CN_59219335_380000_CN96951146/RConn2
  _CN_416989699_380000_CN96951146/RConn3 -- "G_96951146_Centrale_termoelettrica_\"Alessandro_Volta\""/RConn3 -- _CN_59219335_380000_CN96951146/RConn3 -- bus272/LConn1
  Casellina_Calenzano_CN_40634284_380000_CN_139975773_380000/LConn1 -- T_40634284_380000_Calenzano/LConn1 -- Casellina_Calenzano_CN_40634284_380000_CN_41360305_380000/LConn1 -- Calenzano_Suvereto_CN_40634284_380000_CN_107683818_380000/LConn1 -- Bargi___Calenzano_CN_40634284_380000_CN_114931087_380000/LConn1
  Casellina_Calenzano_CN_40634284_380000_CN_139975773_380000/LConn2 -- T_40634284_380000_Calenzano/LConn2 -- Casellina_Calenzano_CN_40634284_380000_CN_41360305_380000/LConn2 -- Calenzano_Suvereto_CN_40634284_380000_CN_107683818_380000/LConn2 -- Bargi___Calenzano_CN_40634284_380000_CN_114931087_380000/LConn2
  Casellina_Calenzano_CN_40634284_380000_CN_139975773_380000/LConn3 -- T_40634284_380000_Calenzano/LConn3 -- Casellina_Calenzano_CN_40634284_380000_CN_41360305_380000/LConn3 -- Calenzano_Suvereto_CN_40634284_380000_CN_107683818_380000/LConn3 -- Bargi___Calenzano_CN_40634284_380000_CN_114931087_380000/LConn3 -- bus273/LConn1
  Casellina_Calenzano_CN_40634284_380000_CN_139975773_380000/RConn1 -- T_139975773_380000_Casellina/LConn1 -- _CN_139975773_380000_CN_140710344_380000/LConn1
  Casellina_Calenzano_CN_40634284_380000_CN_139975773_380000/RConn2 -- T_139975773_380000_Casellina/LConn2 -- _CN_139975773_380000_CN_140710344_380000/LConn2
  Casellina_Calenzano_CN_40634284_380000_CN_139975773_380000/RConn3 -- T_139975773_380000_Casellina/LConn3 -- _CN_139975773_380000_CN_140710344_380000/LConn3 -- bus274/LConn1
  Casellina_Calenzano_CN_40634284_380000_CN_41360305_380000/RConn1 -- T_41360305_380000_Poggio_a_Caiano/LConn1 -- Poggio_a_Caiano___Pian_della_Speranza_CN_83805453_380000_CN_41360305_380000/LConn1
  Casellina_Calenzano_CN_40634284_380000_CN_41360305_380000/RConn2 -- T_41360305_380000_Poggio_a_Caiano/LConn2 -- Poggio_a_Caiano___Pian_della_Speranza_CN_83805453_380000_CN_41360305_380000/LConn2
  Casellina_Calenzano_CN_40634284_380000_CN_41360305_380000/RConn3 -- T_41360305_380000_Poggio_a_Caiano/LConn3 -- Poggio_a_Caiano___Pian_della_Speranza_CN_83805453_380000_CN_41360305_380000/LConn3 -- bus275/LConn1
  Calenzano_Suvereto_CN_40634284_380000_CN_107683818_380000/RConn1 -- T_107683818_380000_Stazione_elettrica_Marginone/LConn1 -- La_Spezia___Marginone_CN_105757794_380000_CN_107683818_380000/LConn1 -- _CN_107681459_380000_CN_107683818_380000/LConn1
  Calenzano_Suvereto_CN_40634284_380000_CN_107683818_380000/RConn2 -- T_107683818_380000_Stazione_elettrica_Marginone/LConn2 -- La_Spezia___Marginone_CN_105757794_380000_CN_107683818_380000/LConn2 -- _CN_107681459_380000_CN_107683818_380000/LConn2
  Calenzano_Suvereto_CN_40634284_380000_CN_107683818_380000/RConn3 -- T_107683818_380000_Stazione_elettrica_Marginone/LConn3 -- La_Spezia___Marginone_CN_105757794_380000_CN_107683818_380000/LConn3 -- bus276/LConn1 -- _CN_107681459_380000_CN_107683818_380000/LConn3
  Bargi___Calenzano_CN_40634284_380000_CN_114931087_380000/RConn1 -- T_114931087_380000_Bargi/LConn1 -- Martignone_Bargi_CN_338453112_380000_CN_114931087_380000/LConn1 -- _CN_114931087_380000_CN259565911/LConn1
  Bargi___Calenzano_CN_40634284_380000_CN_114931087_380000/RConn2 -- T_114931087_380000_Bargi/LConn2 -- Martignone_Bargi_CN_338453112_380000_CN_114931087_380000/LConn2 -- _CN_114931087_380000_CN259565911/LConn2
  Bargi___Calenzano_CN_40634284_380000_CN_114931087_380000/RConn3 -- T_114931087_380000_Bargi/LConn3 -- Martignone_Bargi_CN_338453112_380000_CN_114931087_380000/LConn3 -- _CN_114931087_380000_CN259565911/LConn3 -- bus277/LConn1
  Mercallo___Musignano_CN_72570378_380000_CN_72581705_380000/LConn1 -- T_72570378_380000_Musignano/LConn1 -- _CN_72570378_380000_CN_75604825_380000/LConn1 -- _CN_72570378_380000_CN_72570474_380000/LConn1
  Mercallo___Musignano_CN_72570378_380000_CN_72581705_380000/LConn2 -- T_72570378_380000_Musignano/LConn2 -- _CN_72570378_380000_CN_75604825_380000/LConn2 -- _CN_72570378_380000_CN_72570474_380000/LConn2
  Mercallo___Musignano_CN_72570378_380000_CN_72581705_380000/LConn3 -- T_72570378_380000_Musignano/LConn3 -- _CN_72570378_380000_CN_75604825_380000/LConn3 -- _CN_72570378_380000_CN_72570474_380000/LConn3 -- bus278/LConn1
  Mercallo___Musignano_CN_72570378_380000_CN_72581705_380000/RConn1 -- T_72581705_380000_Mercallo/LConn1 -- Turbigo_Mercallo_CN_72581705_380000_CN_162828577_380000/LConn1
  Mercallo___Musignano_CN_72570378_380000_CN_72581705_380000/RConn2 -- T_72581705_380000_Mercallo/LConn2 -- Turbigo_Mercallo_CN_72581705_380000_CN_162828577_380000/LConn2
  Mercallo___Musignano_CN_72570378_380000_CN_72581705_380000/RConn3 -- T_72581705_380000_Mercallo/LConn3 -- Turbigo_Mercallo_CN_72581705_380000_CN_162828577_380000/LConn3 -- bus279/LConn1
  T_75604825_380000_Roncovalgrande/LConn1 -- _CN_72570378_380000_CN_75604825_380000/RConn1
  T_75604825_380000_Roncovalgrande/LConn2 -- _CN_72570378_380000_CN_75604825_380000/RConn2
  _CN_72570378_380000_CN_75604825_380000/RConn3 -- T_75604825_380000_Roncovalgrande/LConn3 -- bus280/LConn1
  _CN_72570378_380000_CN_72570474_380000/RConn1 -- T_72570474_380000_Cagno/LConn1 -- Cagno_Cislago_CN_72570474_380000_CN_75378894_380000/LConn1
  _CN_72570378_380000_CN_72570474_380000/RConn2 -- T_72570474_380000_Cagno/LConn2 -- Cagno_Cislago_CN_72570474_380000_CN_75378894_380000/LConn2
  _CN_72570378_380000_CN_72570474_380000/RConn3 -- T_72570474_380000_Cagno/LConn3 -- Cagno_Cislago_CN_72570474_380000_CN_75378894_380000/LConn3 -- bus281/LConn1
  _CN_39255054_380000_CN_78066534_380000/LConn1 -- T_39255054_380000_Parma_Vigheffio/LConn1 -- _CN_39255054_380000_CN_93315059_380000/LConn1 -- Parma_Vigheffio_La_Spezia_CN_39255054_380000_CN_105757794_380000/LConn1
  _CN_39255054_380000_CN_78066534_380000/LConn2 -- T_39255054_380000_Parma_Vigheffio/LConn2 -- _CN_39255054_380000_CN_93315059_380000/LConn2 -- Parma_Vigheffio_La_Spezia_CN_39255054_380000_CN_105757794_380000/LConn2
  _CN_39255054_380000_CN_78066534_380000/LConn3 -- T_39255054_380000_Parma_Vigheffio/LConn3 -- _CN_39255054_380000_CN_93315059_380000/LConn3 -- Parma_Vigheffio_La_Spezia_CN_39255054_380000_CN_105757794_380000/LConn3 -- bus282/LConn1
  _CN_39255054_380000_CN_78066534_380000/RConn1 -- T_78066534_380000_Rubiera/LConn1 -- San_Damaso_Martignone_CN_338453112_380000_CN_78066534_380000/LConn1
  _CN_39255054_380000_CN_78066534_380000/RConn2 -- T_78066534_380000_Rubiera/LConn2 -- San_Damaso_Martignone_CN_338453112_380000_CN_78066534_380000/LConn2
  _CN_39255054_380000_CN_78066534_380000/RConn3 -- T_78066534_380000_Rubiera/LConn3 -- San_Damaso_Martignone_CN_338453112_380000_CN_78066534_380000/LConn3 -- bus283/LConn1
  _CN_39255054_380000_CN_93315059_380000/RConn1 -- T_93315059_380000_San_Rocco_Po/LConn1 -- _CN_202271565_380000_CN_93315059_380000/LConn1 -- San_Rocco_Turano_CN_339104227_380000_CN_93315059_380000/LConn1 -- Maleo_San_Rocco_CN_211180338_380000_CN_93315059_380000/LConn1 -- Piacenza_San_Rocco_CN_421827453_380000_CN_93315059_380000/LConn1
  _CN_39255054_380000_CN_93315059_380000/RConn2 -- T_93315059_380000_San_Rocco_Po/LConn2 -- _CN_202271565_380000_CN_93315059_380000/LConn2 -- San_Rocco_Turano_CN_339104227_380000_CN_93315059_380000/LConn2 -- Maleo_San_Rocco_CN_211180338_380000_CN_93315059_380000/LConn2 -- Piacenza_San_Rocco_CN_421827453_380000_CN_93315059_380000/LConn2
  _CN_39255054_380000_CN_93315059_380000/RConn3 -- T_93315059_380000_San_Rocco_Po/LConn3 -- _CN_202271565_380000_CN_93315059_380000/LConn3 -- San_Rocco_Turano_CN_339104227_380000_CN_93315059_380000/LConn3 -- bus284/LConn1 -- Maleo_San_Rocco_CN_211180338_380000_CN_93315059_380000/LConn3 -- Piacenza_San_Rocco_CN_421827453_380000_CN_93315059_380000/LConn3
  Parma_Vigheffio_La_Spezia_CN_39255054_380000_CN_105757794_380000/RConn1 -- T_105757794_380000_La_Spezia/LConn1 -- _CN_105757794_380000_CN116176063/LConn1 -- La_Spezia___Marginone_CN_105757794_380000_CN_107683818_380000/RConn1 -- Vignole_La_Spezia_CN_105757794_380000_CN_100952845_380000/LConn1 -- Acciaiolo_–_Spezia_Stazione_CN_107681459_380000_CN_105757794_380000/LConn1
  Parma_Vigheffio_La_Spezia_CN_39255054_380000_CN_105757794_380000/RConn2 -- T_105757794_380000_La_Spezia/LConn2 -- _CN_105757794_380000_CN116176063/LConn2 -- La_Spezia___Marginone_CN_105757794_380000_CN_107683818_380000/RConn2 -- Vignole_La_Spezia_CN_105757794_380000_CN_100952845_380000/LConn2 -- Acciaiolo_–_Spezia_Stazione_CN_107681459_380000_CN_105757794_380000/LConn2
  Parma_Vigheffio_La_Spezia_CN_39255054_380000_CN_105757794_380000/RConn3 -- T_105757794_380000_La_Spezia/LConn3 -- _CN_105757794_380000_CN116176063/LConn3 -- bus285/LConn1 -- La_Spezia___Marginone_CN_105757794_380000_CN_107683818_380000/RConn3 -- Vignole_La_Spezia_CN_105757794_380000_CN_100952845_380000/LConn3 -- Acciaiolo_–_Spezia_Stazione_CN_107681459_380000_CN_105757794_380000/LConn3
  Maida_Rizziconi_CN_303965869_380000_CN_109993642_380000/LConn1 -- T_303965869_380000_Maida/LConn1 -- Maida_Magisano_CN_303965869_380000_CN_199676823_380000/LConn1
  Maida_Rizziconi_CN_303965869_380000_CN_109993642_380000/LConn2 -- T_303965869_380000_Maida/LConn2 -- Maida_Magisano_CN_303965869_380000_CN_199676823_380000/LConn2
  Maida_Rizziconi_CN_303965869_380000_CN_109993642_380000/LConn3 -- T_303965869_380000_Maida/LConn3 -- Maida_Magisano_CN_303965869_380000_CN_199676823_380000/LConn3 -- bus286/LConn1
  Maida_Rizziconi_CN_303965869_380000_CN_109993642_380000/RConn1 -- T_109993642_380000_Rizziconi/LConn1 -- _CN_109997676_380000_CN_109993642_380000/LConn1 -- Feroleto_Rizziconi_CN_110310021_380000_CN_109993642_380000/LConn1 -- _CN_109993642_380000_CN281858231/LConn1
  Maida_Rizziconi_CN_303965869_380000_CN_109993642_380000/RConn2 -- T_109993642_380000_Rizziconi/LConn2 -- _CN_109997676_380000_CN_109993642_380000/LConn2 -- Feroleto_Rizziconi_CN_110310021_380000_CN_109993642_380000/LConn2 -- _CN_109993642_380000_CN281858231/LConn2
  Maida_Rizziconi_CN_303965869_380000_CN_109993642_380000/RConn3 -- T_109993642_380000_Rizziconi/LConn3 -- _CN_109997676_380000_CN_109993642_380000/LConn3 -- Feroleto_Rizziconi_CN_110310021_380000_CN_109993642_380000/LConn3 -- _CN_109993642_380000_CN281858231/LConn3 -- bus287/LConn1
  Maida_Magisano_CN_303965869_380000_CN_199676823_380000/RConn1 -- T_199676823_380000_Magisano/LConn1 -- Magisano_Scandale_CN_199676823_380000_CN_109756016_380000/LConn1 -- _CN_199675964_380000_CN_199676823_380000/LConn1
  Maida_Magisano_CN_303965869_380000_CN_199676823_380000/RConn2 -- T_199676823_380000_Magisano/LConn2 -- Magisano_Scandale_CN_199676823_380000_CN_109756016_380000/LConn2 -- _CN_199675964_380000_CN_199676823_380000/LConn2
  Maida_Magisano_CN_303965869_380000_CN_199676823_380000/RConn3 -- T_199676823_380000_Magisano/LConn3 -- Magisano_Scandale_CN_199676823_380000_CN_109756016_380000/LConn3 -- bus288/LConn1 -- _CN_199675964_380000_CN_199676823_380000/LConn3
  _CN_98421779_380000_CN98325521/LConn1 -- T_98421779_380000_Trino_Centrale/LConn1 -- Trino_Centrale___Castelnuovo_Scrivia_CN_98421779_380000_CN_98427149_380000/LConn1 -- Rondissone_Trino_2_CN_98421779_380000_CN_74869121_380000/LConn1
  _CN_98421779_380000_CN98325521/LConn2 -- T_98421779_380000_Trino_Centrale/LConn2 -- Trino_Centrale___Castelnuovo_Scrivia_CN_98421779_380000_CN_98427149_380000/LConn2 -- Rondissone_Trino_2_CN_98421779_380000_CN_74869121_380000/LConn2
  _CN_98421779_380000_CN98325521/LConn3 -- T_98421779_380000_Trino_Centrale/LConn3 -- Trino_Centrale___Castelnuovo_Scrivia_CN_98421779_380000_CN_98427149_380000/LConn3 -- bus289/LConn1 -- Rondissone_Trino_2_CN_98421779_380000_CN_74869121_380000/LConn3
  _CN_98421779_380000_CN98325521/RConn1 -- "G_98325521_Centrale_Termoelettrica_\"Galileo_Ferraris\""/RConn1 -- _CN_236661269_380000_CN98325521/LConn1
  _CN_98421779_380000_CN98325521/RConn2 -- "G_98325521_Centrale_Termoelettrica_\"Galileo_Ferraris\""/RConn2 -- _CN_236661269_380000_CN98325521/LConn2
  _CN_98421779_380000_CN98325521/RConn3 -- "G_98325521_Centrale_Termoelettrica_\"Galileo_Ferraris\""/RConn3 -- _CN_236661269_380000_CN98325521/LConn3 -- bus290/LConn1
  Rondissone_Trino_2_CN_98421779_380000_CN_74869121_380000/RConn1 -- T_74869121_380000_Rondissone/LConn1 -- Rondissone_Leini_CN_74869121_380000_CN_105153431_380000/LConn1 -- _CN_105141365_380000_CN_74869121_380000/LConn1 -- Rondissone___Turbigo_CN_162828577_380000_CN_74869121_380000/LConn1 -- Chivasso_Termica___Rondissone_CN_105581403_380000_CN_74869121_380000/LConn1
  Rondissone_Trino_2_CN_98421779_380000_CN_74869121_380000/RConn2 -- T_74869121_380000_Rondissone/LConn2 -- Rondissone_Leini_CN_74869121_380000_CN_105153431_380000/LConn2 -- _CN_105141365_380000_CN_74869121_380000/LConn2 -- Rondissone___Turbigo_CN_162828577_380000_CN_74869121_380000/LConn2 -- Chivasso_Termica___Rondissone_CN_105581403_380000_CN_74869121_380000/LConn2
  Rondissone_Trino_2_CN_98421779_380000_CN_74869121_380000/RConn3 -- T_74869121_380000_Rondissone/LConn3 -- Rondissone_Leini_CN_74869121_380000_CN_105153431_380000/LConn3 -- bus291/LConn1 -- _CN_105141365_380000_CN_74869121_380000/LConn3 -- Rondissone___Turbigo_CN_162828577_380000_CN_74869121_380000/LConn3 -- Chivasso_Termica___Rondissone_CN_105581403_380000_CN_74869121_380000/LConn3
  Trino_Centrale___Castelnuovo_Scrivia_CN_98421779_380000_CN_98427149_380000/RConn1 -- T_98427149_380000_Castelnuovo/LConn1 -- Voghera_Castelnuovo_CN_98901130_380000_CN_98427149_380000/LConn1 -- Vignole_Castelnuovo_CN_100952845_380000_CN_98427149_380000/LConn1
  Trino_Centrale___Castelnuovo_Scrivia_CN_98421779_380000_CN_98427149_380000/RConn2 -- T_98427149_380000_Castelnuovo/LConn2 -- Voghera_Castelnuovo_CN_98901130_380000_CN_98427149_380000/LConn2 -- Vignole_Castelnuovo_CN_100952845_380000_CN_98427149_380000/LConn2
  Trino_Centrale___Castelnuovo_Scrivia_CN_98421779_380000_CN_98427149_380000/RConn3 -- T_98427149_380000_Castelnuovo/LConn3 -- Voghera_Castelnuovo_CN_98901130_380000_CN_98427149_380000/LConn3 -- Vignole_Castelnuovo_CN_100952845_380000_CN_98427149_380000/LConn3 -- bus292/LConn1
  _CN_236661269_380000_CN_202271565_380000/LConn1 -- T_236661269_380000_Lacchiarella/LConn1 -- _CN_236661269_380000_CN98325521/RConn1 -- _CN_236661269_380000_CN_62326314_380000/LConn1
  _CN_236661269_380000_CN_202271565_380000/LConn2 -- T_236661269_380000_Lacchiarella/LConn2 -- _CN_236661269_380000_CN98325521/RConn2 -- _CN_236661269_380000_CN_62326314_380000/LConn2
  _CN_236661269_380000_CN_202271565_380000/LConn3 -- T_236661269_380000_Lacchiarella/LConn3 -- _CN_236661269_380000_CN98325521/RConn3 -- _CN_236661269_380000_CN_62326314_380000/LConn3 -- bus293/LConn1
  _CN_236661269_380000_CN_202271565_380000/RConn1 -- T_202271565_380000_Chignolo_Po/LConn1 -- _CN_211180338_380000_CN_202271565_380000/LConn1 -- _CN_107438024_380000_CN_202271565_380000/LConn1 -- _CN_202271565_380000_CN_93315059_380000/RConn1
  _CN_236661269_380000_CN_202271565_380000/RConn2 -- T_202271565_380000_Chignolo_Po/LConn2 -- _CN_211180338_380000_CN_202271565_380000/LConn2 -- _CN_107438024_380000_CN_202271565_380000/LConn2 -- _CN_202271565_380000_CN_93315059_380000/RConn2
  _CN_236661269_380000_CN_202271565_380000/RConn3 -- T_202271565_380000_Chignolo_Po/LConn3 -- _CN_211180338_380000_CN_202271565_380000/LConn3 -- _CN_107438024_380000_CN_202271565_380000/LConn3 -- _CN_202271565_380000_CN_93315059_380000/RConn3 -- bus294/LConn1
  _CN_236661269_380000_CN_62326314_380000/RConn1 -- T_62326314_380000_Baggio/LConn1 -- _CN_162828577_380000_CN_62326314_380000/LConn1 -- _CN_189612607_380000_CN_62326314_380000/LConn1 -- _CN_93038661_380000_CN_62326314_380000/LConn1
  _CN_236661269_380000_CN_62326314_380000/RConn2 -- T_62326314_380000_Baggio/LConn2 -- _CN_162828577_380000_CN_62326314_380000/LConn2 -- _CN_189612607_380000_CN_62326314_380000/LConn2 -- _CN_93038661_380000_CN_62326314_380000/LConn2
  _CN_236661269_380000_CN_62326314_380000/RConn3 -- T_62326314_380000_Baggio/LConn3 -- _CN_162828577_380000_CN_62326314_380000/LConn3 -- bus295/LConn1 -- _CN_189612607_380000_CN_62326314_380000/LConn3 -- _CN_93038661_380000_CN_62326314_380000/LConn3
  Castellaneta_Taranto_Nord_CN_103381531_380000_CN_338760116_380000/LConn1 -- T_103381531_380000_Taranto_Nord/LConn1 -- Brindisi_Taranto_nord_CN_103381531_380000_CN_60919237_380000/RConn1 -- Galatina_Taranto_nord_CN_103381531_380000_CN_103386958_380000/LConn1
  Castellaneta_Taranto_Nord_CN_103381531_380000_CN_338760116_380000/LConn2 -- T_103381531_380000_Taranto_Nord/LConn2 -- Brindisi_Taranto_nord_CN_103381531_380000_CN_60919237_380000/RConn2 -- Galatina_Taranto_nord_CN_103381531_380000_CN_103386958_380000/LConn2
  Castellaneta_Taranto_Nord_CN_103381531_380000_CN_338760116_380000/LConn3 -- T_103381531_380000_Taranto_Nord/LConn3 -- Brindisi_Taranto_nord_CN_103381531_380000_CN_60919237_380000/RConn3 -- Galatina_Taranto_nord_CN_103381531_380000_CN_103386958_380000/LConn3 -- bus296/LConn1
  Castellaneta_Taranto_Nord_CN_103381531_380000_CN_338760116_380000/RConn1 -- T_338760116_380000_Castellaneta/LConn1 -- Castellaneta_Matera_CN_103306951_380000_CN_338760116_380000/LConn1
  Castellaneta_Taranto_Nord_CN_103381531_380000_CN_338760116_380000/RConn2 -- T_338760116_380000_Castellaneta/LConn2 -- Castellaneta_Matera_CN_103306951_380000_CN_338760116_380000/LConn2
  Castellaneta_Taranto_Nord_CN_103381531_380000_CN_338760116_380000/RConn3 -- T_338760116_380000_Castellaneta/LConn3 -- Castellaneta_Matera_CN_103306951_380000_CN_338760116_380000/LConn3 -- bus297/LConn1
  Galatina_Taranto_nord_CN_103381531_380000_CN_103386958_380000/RConn1 -- T_103386958_380000_Galatina/LConn1 -- Galatina_Brindisi_sud_CN_60888331_380000_CN_103386958_380000/LConn1
  Galatina_Taranto_nord_CN_103381531_380000_CN_103386958_380000/RConn2 -- T_103386958_380000_Galatina/LConn2 -- Galatina_Brindisi_sud_CN_60888331_380000_CN_103386958_380000/LConn2
  Galatina_Taranto_nord_CN_103381531_380000_CN_103386958_380000/RConn3 -- T_103386958_380000_Galatina/LConn3 -- Galatina_Brindisi_sud_CN_60888331_380000_CN_103386958_380000/LConn3 -- bus298/LConn1
  Dugale_Ostiglia_CN_82078641_380000_CN_59556712_380000/LConn1 -- T_82078641_380000_Ostiglia/LConn1 -- _CN_82078641_380000_CN_421827452_380000/LConn1 -- Mantova_Ostiglia_CN_82078641_380000_CN_116697005_380000/LConn1 -- Ostiglia_Ferrara_Nord_CN_82078641_380000_CN_82084013_380000/LConn1 -- Ostiglia_Sermide_CN_82078641_380000_CN_82084019_380000/LConn1
  Dugale_Ostiglia_CN_82078641_380000_CN_59556712_380000/LConn2 -- T_82078641_380000_Ostiglia/LConn2 -- _CN_82078641_380000_CN_421827452_380000/LConn2 -- Mantova_Ostiglia_CN_82078641_380000_CN_116697005_380000/LConn2 -- Ostiglia_Ferrara_Nord_CN_82078641_380000_CN_82084013_380000/LConn2 -- Ostiglia_Sermide_CN_82078641_380000_CN_82084019_380000/LConn2
  Dugale_Ostiglia_CN_82078641_380000_CN_59556712_380000/LConn3 -- T_82078641_380000_Ostiglia/LConn3 -- _CN_82078641_380000_CN_421827452_380000/LConn3 -- Mantova_Ostiglia_CN_82078641_380000_CN_116697005_380000/LConn3 -- bus299/LConn1 -- Ostiglia_Ferrara_Nord_CN_82078641_380000_CN_82084013_380000/LConn3 -- Ostiglia_Sermide_CN_82078641_380000_CN_82084019_380000/LConn3
  Dugale_Ostiglia_CN_82078641_380000_CN_59556712_380000/RConn1 -- T_59556712_380000_Dugale/LConn1 -- Dugale_Nogarole_Rocca_CN_155791516_380000_CN_59556712_380000/LConn1 -- _CN_64942789_380000_CN_59556712_380000/LConn1 -- _CN_59366523_380000_CN_59556712_380000/LConn1
  Dugale_Ostiglia_CN_82078641_380000_CN_59556712_380000/RConn2 -- T_59556712_380000_Dugale/LConn2 -- Dugale_Nogarole_Rocca_CN_155791516_380000_CN_59556712_380000/LConn2 -- _CN_64942789_380000_CN_59556712_380000/LConn2 -- _CN_59366523_380000_CN_59556712_380000/LConn2
  Dugale_Ostiglia_CN_82078641_380000_CN_59556712_380000/RConn3 -- T_59556712_380000_Dugale/LConn3 -- Dugale_Nogarole_Rocca_CN_155791516_380000_CN_59556712_380000/LConn3 -- _CN_64942789_380000_CN_59556712_380000/LConn3 -- bus300/LConn1 -- _CN_59366523_380000_CN_59556712_380000/LConn3
  Ostiglia_Sermide_CN_82078641_380000_CN_82084019_380000/RConn1 -- T_82084019_380000_Sermide/LConn1 -- Martignone___Sermide_CN_338453112_380000_CN_82084019_380000/LConn1
  Ostiglia_Sermide_CN_82078641_380000_CN_82084019_380000/RConn2 -- T_82084019_380000_Sermide/LConn2 -- Martignone___Sermide_CN_338453112_380000_CN_82084019_380000/LConn2
  Ostiglia_Sermide_CN_82078641_380000_CN_82084019_380000/RConn3 -- T_82084019_380000_Sermide/LConn3 -- Martignone___Sermide_CN_338453112_380000_CN_82084019_380000/LConn3 -- bus301/LConn1
  Ostiglia_Ferrara_Nord_CN_82078641_380000_CN_82084013_380000/RConn1 -- T_82084013_380000_Ferrara_Nord/LConn1 -- Focomorto_Ferrara_Nord_CN_363469921_380000_CN_82084013_380000/LConn1 -- _CN_365525159_380000_CN_82084013_380000/LConn1
  Ostiglia_Ferrara_Nord_CN_82078641_380000_CN_82084013_380000/RConn2 -- T_82084013_380000_Ferrara_Nord/LConn2 -- Focomorto_Ferrara_Nord_CN_363469921_380000_CN_82084013_380000/LConn2 -- _CN_365525159_380000_CN_82084013_380000/LConn2
  Ostiglia_Ferrara_Nord_CN_82078641_380000_CN_82084013_380000/RConn3 -- T_82084013_380000_Ferrara_Nord/LConn3 -- Focomorto_Ferrara_Nord_CN_363469921_380000_CN_82084013_380000/LConn3 -- _CN_365525159_380000_CN_82084013_380000/LConn3 -- bus302/LConn1
  T_421827452_380000_Ostiglia_centrale/LConn1 -- _CN_82078641_380000_CN_421827452_380000/RConn1
  T_421827452_380000_Ostiglia_centrale/LConn2 -- _CN_82078641_380000_CN_421827452_380000/RConn2
  _CN_82078641_380000_CN_421827452_380000/RConn3 -- T_421827452_380000_Ostiglia_centrale/LConn3 -- bus303/LConn1
  Mantova_Ostiglia_CN_82078641_380000_CN_116697005_380000/RConn1 -- T_116697005_380000_Mantova/LConn1 -- Flero_Mantova_CN_58440884_380000_CN_116697005_380000/LConn1 -- _CN_116697005_380000_CN_116912085_380000/LConn1
  Mantova_Ostiglia_CN_82078641_380000_CN_116697005_380000/RConn2 -- T_116697005_380000_Mantova/LConn2 -- Flero_Mantova_CN_58440884_380000_CN_116697005_380000/LConn2 -- _CN_116697005_380000_CN_116912085_380000/LConn2
  Mantova_Ostiglia_CN_82078641_380000_CN_116697005_380000/RConn3 -- T_116697005_380000_Mantova/LConn3 -- Flero_Mantova_CN_58440884_380000_CN_116697005_380000/LConn3 -- _CN_116697005_380000_CN_116912085_380000/LConn3 -- bus304/LConn1
  T_149997403_380000_Eni_Power/LConn1 -- Ravenna_Canala_Enipower_CN_149997403_380000_CN_81938081_380000/LConn1
  T_149997403_380000_Eni_Power/LConn2 -- Ravenna_Canala_Enipower_CN_149997403_380000_CN_81938081_380000/LConn2
  Ravenna_Canala_Enipower_CN_149997403_380000_CN_81938081_380000/LConn3 -- T_149997403_380000_Eni_Power/LConn3 -- bus305/LConn1
  Ravenna_Canala_Enipower_CN_149997403_380000_CN_81938081_380000/RConn1 -- "T_81938081_380000_Stazione_elettrica_\"Ravenna_Canala\""/LConn1 -- Focomorto_Ravenna_Canala_CN_363469921_380000_CN_81938081_380000/LConn1 -- Porto_Tolle_Ravenna_Canala_CN_81938081_380000_CN_81929591_380000/LConn1 -- Porto_Tolle_Ravenna_Canala_CN_81938081_380000_CN_81931074_380000/LConn1 -- Centrale_Teodora___Ravenna_Canala_CN_81938081_380000_CN_158739183_380000/LConn1 -- _CN_81938081_380000_CN_74943205_380000/LConn1
  Ravenna_Canala_Enipower_CN_149997403_380000_CN_81938081_380000/RConn2 -- "T_81938081_380000_Stazione_elettrica_\"Ravenna_Canala\""/LConn2 -- Focomorto_Ravenna_Canala_CN_363469921_380000_CN_81938081_380000/LConn2 -- Porto_Tolle_Ravenna_Canala_CN_81938081_380000_CN_81929591_380000/LConn2 -- Porto_Tolle_Ravenna_Canala_CN_81938081_380000_CN_81931074_380000/LConn2 -- Centrale_Teodora___Ravenna_Canala_CN_81938081_380000_CN_158739183_380000/LConn2 -- _CN_81938081_380000_CN_74943205_380000/LConn2
  Ravenna_Canala_Enipower_CN_149997403_380000_CN_81938081_380000/RConn3 -- "T_81938081_380000_Stazione_elettrica_\"Ravenna_Canala\""/LConn3 -- Focomorto_Ravenna_Canala_CN_363469921_380000_CN_81938081_380000/LConn3 -- Porto_Tolle_Ravenna_Canala_CN_81938081_380000_CN_81929591_380000/LConn3 -- Porto_Tolle_Ravenna_Canala_CN_81938081_380000_CN_81931074_380000/LConn3 -- Centrale_Teodora___Ravenna_Canala_CN_81938081_380000_CN_158739183_380000/LConn3 -- _CN_81938081_380000_CN_74943205_380000/LConn3 -- bus306/LConn1
  _CN_75947556_380000_CN_133601335_380000/LConn1 -- T_75947556_380000_Ciserano/LConn1 -- _CN_75947556_380000_CN_162960205_380000/LConn1
  _CN_75947556_380000_CN_133601335_380000/LConn2 -- T_75947556_380000_Ciserano/LConn2 -- _CN_75947556_380000_CN_162960205_380000/LConn2
  _CN_75947556_380000_CN_133601335_380000/LConn3 -- T_75947556_380000_Ciserano/LConn3 -- _CN_75947556_380000_CN_162960205_380000/LConn3 -- bus307/LConn1
  T_133601335_380000_Cassano/LConn1 -- _CN_75947556_380000_CN_133601335_380000/RConn1
  T_133601335_380000_Cassano/LConn2 -- _CN_75947556_380000_CN_133601335_380000/RConn2
  _CN_75947556_380000_CN_133601335_380000/RConn3 -- T_133601335_380000_Cassano/LConn3 -- bus308/LConn1
  _CN_75947556_380000_CN_162960205_380000/RConn1 -- T_162960205_380000_Tavazzano_Centrale/LConn1 -- Turano_Tavazzano_CN_162960205_380000_CN_339104227_380000/LConn1 -- _CN_68299044_380000_CN_162960205_380000/LConn1
  _CN_75947556_380000_CN_162960205_380000/RConn2 -- T_162960205_380000_Tavazzano_Centrale/LConn2 -- Turano_Tavazzano_CN_162960205_380000_CN_339104227_380000/LConn2 -- _CN_68299044_380000_CN_162960205_380000/LConn2
  _CN_75947556_380000_CN_162960205_380000/RConn3 -- T_162960205_380000_Tavazzano_Centrale/LConn3 -- Turano_Tavazzano_CN_162960205_380000_CN_339104227_380000/LConn3 -- bus309/LConn1 -- _CN_68299044_380000_CN_162960205_380000/LConn3
  Monfalcone_Termoelettrica___Redipuglia_CN_41892273_380000_CN_60725875_380000/LConn1 -- T_41892273_380000_Redipuglia/LConn1 -- Planais___Redipuglia_CN_41892273_380000_CN_58992998_380000/LConn1 -- Planais___Redipuglia_CN_41892273_380000_CN_59026315_380000/LConn1
  Monfalcone_Termoelettrica___Redipuglia_CN_41892273_380000_CN_60725875_380000/LConn2 -- T_41892273_380000_Redipuglia/LConn2 -- Planais___Redipuglia_CN_41892273_380000_CN_58992998_380000/LConn2 -- Planais___Redipuglia_CN_41892273_380000_CN_59026315_380000/LConn2
  Monfalcone_Termoelettrica___Redipuglia_CN_41892273_380000_CN_60725875_380000/LConn3 -- T_41892273_380000_Redipuglia/LConn3 -- Planais___Redipuglia_CN_41892273_380000_CN_58992998_380000/LConn3 -- Planais___Redipuglia_CN_41892273_380000_CN_59026315_380000/LConn3 -- bus310/LConn1
  T_60725875_380000_Monfalcone_sezione_1_400/LConn1 -- Monfalcone_Termoelettrica___Redipuglia_CN_41892273_380000_CN_60725875_380000/RConn1
  T_60725875_380000_Monfalcone_sezione_1_400/LConn2 -- Monfalcone_Termoelettrica___Redipuglia_CN_41892273_380000_CN_60725875_380000/RConn2
  Monfalcone_Termoelettrica___Redipuglia_CN_41892273_380000_CN_60725875_380000/RConn3 -- T_60725875_380000_Monfalcone_sezione_1_400/LConn3 -- bus311/LConn1
  Planais___Redipuglia_CN_41892273_380000_CN_58992998_380000/RConn1 -- T_58992998_380000_Planais/LConn1 -- Torviscosa___Planais_CN_59462715_380000_CN_58992998_380000/LConn1 -- Planais___Udine_Ovest_CN_58992998_380000_CN_59462263_380000/LConn1
  Planais___Redipuglia_CN_41892273_380000_CN_58992998_380000/RConn2 -- T_58992998_380000_Planais/LConn2 -- Torviscosa___Planais_CN_59462715_380000_CN_58992998_380000/LConn2 -- Planais___Udine_Ovest_CN_58992998_380000_CN_59462263_380000/LConn2
  Planais___Redipuglia_CN_41892273_380000_CN_58992998_380000/RConn3 -- T_58992998_380000_Planais/LConn3 -- Torviscosa___Planais_CN_59462715_380000_CN_58992998_380000/LConn3 -- Planais___Udine_Ovest_CN_58992998_380000_CN_59462263_380000/LConn3 -- bus312/LConn1
  Planais___Redipuglia_CN_41892273_380000_CN_59026315_380000/RConn1 -- T_59026315_380000_Salgareda/LConn1 -- _CN_84301904_380000_CN_59026315_380000/LConn1
  Planais___Redipuglia_CN_41892273_380000_CN_59026315_380000/RConn2 -- T_59026315_380000_Salgareda/LConn2 -- _CN_84301904_380000_CN_59026315_380000/LConn2
  Planais___Redipuglia_CN_41892273_380000_CN_59026315_380000/RConn3 -- T_59026315_380000_Salgareda/LConn3 -- _CN_84301904_380000_CN_59026315_380000/LConn3 -- bus313/LConn1
  _CN_36873258_380000_CN61940739/LConn1 -- T_36873258_380000_Candia/LConn1 -- _CN_36873258_380000_CN_61626687_380000/LConn1 -- _CN_36873258_380000_CN_74943205_380000/LConn1
  _CN_36873258_380000_CN61940739/LConn2 -- T_36873258_380000_Candia/LConn2 -- _CN_36873258_380000_CN_61626687_380000/LConn2 -- _CN_36873258_380000_CN_74943205_380000/LConn2
  _CN_36873258_380000_CN61940739/LConn3 -- T_36873258_380000_Candia/LConn3 -- _CN_36873258_380000_CN_61626687_380000/LConn3 -- _CN_36873258_380000_CN_74943205_380000/LConn3 -- bus314/LConn1
  G_61940739_/RConn1 -- _CN_36873258_380000_CN61940739/RConn1
  G_61940739_/RConn2 -- _CN_36873258_380000_CN61940739/RConn2
  _CN_36873258_380000_CN61940739/RConn3 -- G_61940739_/RConn3 -- bus315/LConn1
  _CN_36873258_380000_CN_61626687_380000/RConn1 -- T_61626687_380000_Teramo/LConn1 -- Teramo_San_Giacomo_380_CN_96190189_380000_CN_61626687_380000/LConn1 -- Teramo_Villanova_CN_61375111_380000_CN_61626687_380000/RConn1
  _CN_36873258_380000_CN_61626687_380000/RConn2 -- T_61626687_380000_Teramo/LConn2 -- Teramo_San_Giacomo_380_CN_96190189_380000_CN_61626687_380000/LConn2 -- Teramo_Villanova_CN_61375111_380000_CN_61626687_380000/RConn2
  _CN_36873258_380000_CN_61626687_380000/RConn3 -- T_61626687_380000_Teramo/LConn3 -- Teramo_San_Giacomo_380_CN_96190189_380000_CN_61626687_380000/LConn3 -- bus316/LConn1 -- Teramo_Villanova_CN_61375111_380000_CN_61626687_380000/RConn3
  _CN_36873258_380000_CN_74943205_380000/RConn1 -- T_74943205_380000_Fano_Entroterra/LConn1 -- _CN_81938081_380000_CN_74943205_380000/RConn1 -- _CN_74943205_380000_CN_143585004_380000/LConn1
  _CN_36873258_380000_CN_74943205_380000/RConn2 -- T_74943205_380000_Fano_Entroterra/LConn2 -- _CN_81938081_380000_CN_74943205_380000/RConn2 -- _CN_74943205_380000_CN_143585004_380000/LConn2
  _CN_36873258_380000_CN_74943205_380000/RConn3 -- T_74943205_380000_Fano_Entroterra/LConn3 -- _CN_81938081_380000_CN_74943205_380000/RConn3 -- _CN_74943205_380000_CN_143585004_380000/LConn3 -- bus317/LConn1
  _CN_110330925_380000_CN_110310021_380000/LConn1 -- T_110330925_380000_Altomonte_Centrale/LConn1 -- _CN_110330925_380000_CN_108020416_380000/LConn1
  _CN_110330925_380000_CN_110310021_380000/LConn2 -- T_110330925_380000_Altomonte_Centrale/LConn2 -- _CN_110330925_380000_CN_108020416_380000/LConn2
  _CN_110330925_380000_CN_110310021_380000/LConn3 -- T_110330925_380000_Altomonte_Centrale/LConn3 -- _CN_110330925_380000_CN_108020416_380000/LConn3 -- bus318/LConn1
  _CN_110330925_380000_CN_110310021_380000/RConn1 -- T_110310021_380000_Stazione_Elettrica_di_Feroleto/LConn1 -- Feroleto_Rizziconi_CN_110310021_380000_CN_109993642_380000/RConn1
  _CN_110330925_380000_CN_110310021_380000/RConn2 -- T_110310021_380000_Stazione_Elettrica_di_Feroleto/LConn2 -- Feroleto_Rizziconi_CN_110310021_380000_CN_109993642_380000/RConn2
  _CN_110330925_380000_CN_110310021_380000/RConn3 -- T_110310021_380000_Stazione_Elettrica_di_Feroleto/LConn3 -- Feroleto_Rizziconi_CN_110310021_380000_CN_109993642_380000/RConn3 -- bus319/LConn1
  _CN_110330925_380000_CN_108020416_380000/RConn1 -- T_108020416_380000_Laino/LConn1 -- _CN_85196861_380000_CN_108020416_380000/LConn1 -- _CN_338790588_380000_CN_108020416_380000/LConn1 -- _CN_108020416_380000_CN_109588422_380000/LConn1
  _CN_110330925_380000_CN_108020416_380000/RConn2 -- T_108020416_380000_Laino/LConn2 -- _CN_85196861_380000_CN_108020416_380000/LConn2 -- _CN_338790588_380000_CN_108020416_380000/LConn2 -- _CN_108020416_380000_CN_109588422_380000/LConn2
  _CN_110330925_380000_CN_108020416_380000/RConn3 -- T_108020416_380000_Laino/LConn3 -- _CN_85196861_380000_CN_108020416_380000/LConn3 -- _CN_338790588_380000_CN_108020416_380000/LConn3 -- _CN_108020416_380000_CN_109588422_380000/LConn3 -- bus320/LConn1
  _CN_338792752_380000_CN_418565264_380000/LConn1 -- T_338792752_380000_San_Severo/LConn1 -- Foggia_San_Severo_CN_338792752_380000_CN_418565263_380000/LConn1 -- Larino_San_Severo_CN_338792752_380000_CN_60235685_380000/LConn1
  _CN_338792752_380000_CN_418565264_380000/LConn2 -- T_338792752_380000_San_Severo/LConn2 -- Foggia_San_Severo_CN_338792752_380000_CN_418565263_380000/LConn2 -- Larino_San_Severo_CN_338792752_380000_CN_60235685_380000/LConn2
  _CN_338792752_380000_CN_418565264_380000/LConn3 -- T_338792752_380000_San_Severo/LConn3 -- Foggia_San_Severo_CN_338792752_380000_CN_418565263_380000/LConn3 -- bus321/LConn1 -- Larino_San_Severo_CN_338792752_380000_CN_60235685_380000/LConn3
  T_418565264_380000_Ratino_centrale/LConn1 -- _CN_338792752_380000_CN_418565264_380000/RConn1
  T_418565264_380000_Ratino_centrale/LConn2 -- _CN_338792752_380000_CN_418565264_380000/RConn2
  _CN_338792752_380000_CN_418565264_380000/RConn3 -- T_418565264_380000_Ratino_centrale/LConn3 -- bus322/LConn1
  Larino_San_Severo_CN_338792752_380000_CN_60235685_380000/RConn1 -- T_60235685_380000_Larino/LConn1 -- Gissi_Larino_CN_60616350_380000_CN_60235685_380000/LConn1 -- _CN_411026199_380000_CN_60235685_380000/LConn1
  Larino_San_Severo_CN_338792752_380000_CN_60235685_380000/RConn2 -- T_60235685_380000_Larino/LConn2 -- Gissi_Larino_CN_60616350_380000_CN_60235685_380000/LConn2 -- _CN_411026199_380000_CN_60235685_380000/LConn2
  Larino_San_Severo_CN_338792752_380000_CN_60235685_380000/RConn3 -- T_60235685_380000_Larino/LConn3 -- Gissi_Larino_CN_60616350_380000_CN_60235685_380000/LConn3 -- bus323/LConn1 -- _CN_411026199_380000_CN_60235685_380000/LConn3
  Foggia_San_Severo_CN_338792752_380000_CN_418565263_380000/RConn1 -- T_418565263_380000_Foggia/LConn1 -- Andria_Foggia_CN_418565263_380000_CN_126203383_380000/LConn1 -- _CN_418565263_380000_CN_209982720_380000/LConn1 -- _CN_418565263_380000_CN_338795626_380000/LConn1 -- Foggia_Palo_del_Colle_CN_418565263_380000_CN_146791061_380000/RConn1
  Foggia_San_Severo_CN_338792752_380000_CN_418565263_380000/RConn2 -- T_418565263_380000_Foggia/LConn2 -- Andria_Foggia_CN_418565263_380000_CN_126203383_380000/LConn2 -- _CN_418565263_380000_CN_209982720_380000/LConn2 -- _CN_418565263_380000_CN_338795626_380000/LConn2 -- Foggia_Palo_del_Colle_CN_418565263_380000_CN_146791061_380000/RConn2
  Foggia_San_Severo_CN_338792752_380000_CN_418565263_380000/RConn3 -- T_418565263_380000_Foggia/LConn3 -- Andria_Foggia_CN_418565263_380000_CN_126203383_380000/LConn3 -- bus324/LConn1 -- _CN_418565263_380000_CN_209982720_380000/LConn3 -- _CN_418565263_380000_CN_338795626_380000/LConn3 -- Foggia_Palo_del_Colle_CN_418565263_380000_CN_146791061_380000/RConn3
  _CN_107681459_380000_CN_107683818_380000/RConn1 -- T_107681459_380000_Acciaiolo/LConn1 -- Acciaiolo_–_Spezia_Stazione_CN_107681459_380000_CN_105757794_380000/RConn1 -- Rosignano_Acciaiolo_CN_107681459_380000_CN_116240715_380000/LConn1
  _CN_107681459_380000_CN_107683818_380000/RConn2 -- T_107681459_380000_Acciaiolo/LConn2 -- Acciaiolo_–_Spezia_Stazione_CN_107681459_380000_CN_105757794_380000/RConn2 -- Rosignano_Acciaiolo_CN_107681459_380000_CN_116240715_380000/LConn2
  _CN_107681459_380000_CN_107683818_380000/RConn3 -- T_107681459_380000_Acciaiolo/LConn3 -- Acciaiolo_–_Spezia_Stazione_CN_107681459_380000_CN_105757794_380000/RConn3 -- Rosignano_Acciaiolo_CN_107681459_380000_CN_116240715_380000/LConn3 -- bus325/LConn1
  Rosignano_Acciaiolo_CN_107681459_380000_CN_116240715_380000/RConn1 -- T_116240715_380000_Roselectra/LConn1 -- _CN_116240715_380000_CN_414663585_380000/LConn1
  Rosignano_Acciaiolo_CN_107681459_380000_CN_116240715_380000/RConn2 -- T_116240715_380000_Roselectra/LConn2 -- _CN_116240715_380000_CN_414663585_380000/LConn2
  Rosignano_Acciaiolo_CN_107681459_380000_CN_116240715_380000/RConn3 -- T_116240715_380000_Roselectra/LConn3 -- _CN_116240715_380000_CN_414663585_380000/LConn3 -- bus326/LConn1
  _CN_157912118_380000_CN_109997676_380000/LConn1 -- T_157912118_380000_Stazione_Elettrica_Paradiso/LConn1 -- Elettrodotto_Sorgente___Paradiso_CN_157912118_380000_CN_110138220_380000/LConn1
  _CN_157912118_380000_CN_109997676_380000/LConn2 -- T_157912118_380000_Stazione_Elettrica_Paradiso/LConn2 -- Elettrodotto_Sorgente___Paradiso_CN_157912118_380000_CN_110138220_380000/LConn2
  _CN_157912118_380000_CN_109997676_380000/LConn3 -- T_157912118_380000_Stazione_Elettrica_Paradiso/LConn3 -- Elettrodotto_Sorgente___Paradiso_CN_157912118_380000_CN_110138220_380000/LConn3 -- bus327/LConn1
  _CN_157912118_380000_CN_109997676_380000/RConn1 -- T_109997676_380000_Bolano/LConn1 -- _CN_109997676_380000_CN_109993642_380000/RConn1
  _CN_157912118_380000_CN_109997676_380000/RConn2 -- T_109997676_380000_Bolano/LConn2 -- _CN_109997676_380000_CN_109993642_380000/RConn2
  _CN_157912118_380000_CN_109997676_380000/RConn3 -- T_109997676_380000_Bolano/LConn3 -- _CN_109997676_380000_CN_109993642_380000/RConn3 -- bus328/LConn1
  Elettrodotto_Sorgente___Paradiso_CN_157912118_380000_CN_110138220_380000/RConn1 -- T_110138220_380000_Sorgente/LConn1 -- Elettrodotto_Sorgente___Paternò_CN_110138220_380000_CN_61157826_380000/LConn1
  Elettrodotto_Sorgente___Paradiso_CN_157912118_380000_CN_110138220_380000/RConn2 -- T_110138220_380000_Sorgente/LConn2 -- Elettrodotto_Sorgente___Paternò_CN_110138220_380000_CN_61157826_380000/LConn2
  Elettrodotto_Sorgente___Paradiso_CN_157912118_380000_CN_110138220_380000/RConn3 -- T_110138220_380000_Sorgente/LConn3 -- Elettrodotto_Sorgente___Paternò_CN_110138220_380000_CN_61157826_380000/LConn3 -- bus329/LConn1
  T_59462715_380000_Torviscosa_Edison/LConn1 -- Torviscosa___Planais_CN_59462715_380000_CN_58992998_380000/RConn1
  T_59462715_380000_Torviscosa_Edison/LConn2 -- Torviscosa___Planais_CN_59462715_380000_CN_58992998_380000/RConn2
  Torviscosa___Planais_CN_59462715_380000_CN_58992998_380000/RConn3 -- T_59462715_380000_Torviscosa_Edison/LConn3 -- bus330/LConn1
  T_199675964_380000_Simeri_Crichi/LConn1 -- _CN_199675964_380000_CN_199676823_380000/RConn1
  T_199675964_380000_Simeri_Crichi/LConn2 -- _CN_199675964_380000_CN_199676823_380000/RConn2
  _CN_199675964_380000_CN_199676823_380000/RConn3 -- T_199675964_380000_Simeri_Crichi/LConn3 -- bus331/LConn1
  _CN_85196861_380000_CN_108020416_380000/RConn1 -- T_85196861_380000_Montecorvino/LConn1 -- Montecorvino_Santa_Sofia_CN_85196861_380000_CN_84696559_380000/LConn1
  _CN_85196861_380000_CN_108020416_380000/RConn2 -- T_85196861_380000_Montecorvino/LConn2 -- Montecorvino_Santa_Sofia_CN_85196861_380000_CN_84696559_380000/LConn2
  _CN_85196861_380000_CN_108020416_380000/RConn3 -- T_85196861_380000_Montecorvino/LConn3 -- Montecorvino_Santa_Sofia_CN_85196861_380000_CN_84696559_380000/LConn3 -- bus332/LConn1
  Montecorvino_Santa_Sofia_CN_85196861_380000_CN_84696559_380000/RConn1 -- T_84696559_380000_Santa_Sofia/LConn1 -- _CN_93860115_380000_CN_84696559_380000/LConn1 -- _CN_257351439_380000_CN_84696559_380000/LConn1 -- _CN_114661587_380000_CN_84696559_380000/LConn1
  Montecorvino_Santa_Sofia_CN_85196861_380000_CN_84696559_380000/RConn2 -- T_84696559_380000_Santa_Sofia/LConn2 -- _CN_93860115_380000_CN_84696559_380000/LConn2 -- _CN_257351439_380000_CN_84696559_380000/LConn2 -- _CN_114661587_380000_CN_84696559_380000/LConn2
  Montecorvino_Santa_Sofia_CN_85196861_380000_CN_84696559_380000/RConn3 -- T_84696559_380000_Santa_Sofia/LConn3 -- _CN_93860115_380000_CN_84696559_380000/LConn3 -- bus333/LConn1 -- _CN_257351439_380000_CN_84696559_380000/LConn3 -- _CN_114661587_380000_CN_84696559_380000/LConn3
  _CN_189612607_380000_CN_62326314_380000/RConn1 -- T_189612607_380000_Rho/LConn1 -- _CN_189612607_380000_CN_74677138_380000/LConn1 -- _CN_189612607_380000_CN_34157795_380000/LConn1
  _CN_189612607_380000_CN_62326314_380000/RConn2 -- T_189612607_380000_Rho/LConn2 -- _CN_189612607_380000_CN_74677138_380000/LConn2 -- _CN_189612607_380000_CN_34157795_380000/LConn2
  _CN_189612607_380000_CN_62326314_380000/RConn3 -- T_189612607_380000_Rho/LConn3 -- _CN_189612607_380000_CN_74677138_380000/LConn3 -- _CN_189612607_380000_CN_34157795_380000/LConn3 -- bus334/LConn1
  _CN_189612607_380000_CN_74677138_380000/RConn1 -- T_74677138_380000_Bovisio/LConn1 -- Bovisio_Brugherio_CN_68299044_380000_CN_74677138_380000/LConn1 -- _CN_152597636_380000_CN_74677138_380000/LConn1 -- Bovisio_Cislago_CN_75378894_380000_CN_74677138_380000/LConn1
  _CN_189612607_380000_CN_74677138_380000/RConn2 -- T_74677138_380000_Bovisio/LConn2 -- Bovisio_Brugherio_CN_68299044_380000_CN_74677138_380000/LConn2 -- _CN_152597636_380000_CN_74677138_380000/LConn2 -- Bovisio_Cislago_CN_75378894_380000_CN_74677138_380000/LConn2
  _CN_189612607_380000_CN_74677138_380000/RConn3 -- T_74677138_380000_Bovisio/LConn3 -- Bovisio_Brugherio_CN_68299044_380000_CN_74677138_380000/LConn3 -- bus335/LConn1 -- _CN_152597636_380000_CN_74677138_380000/LConn3 -- Bovisio_Cislago_CN_75378894_380000_CN_74677138_380000/LConn3
  T_34157795_380000_Ospiate/LConn1 -- _CN_189612607_380000_CN_34157795_380000/RConn1
  T_34157795_380000_Ospiate/LConn2 -- _CN_189612607_380000_CN_34157795_380000/RConn2
  _CN_189612607_380000_CN_34157795_380000/RConn3 -- T_34157795_380000_Ospiate/LConn3 -- bus336/LConn1
  _CN_93038661_380000_CN402288342/LConn1 -- T_93038661_380000_Pieve_Albignola/LConn1 -- _CN_93038661_380000_CN_62326314_380000/RConn1 -- Pieve_Albignola_Voghera_CN_93038661_380000_CN_98901130_380000/LConn1
  _CN_93038661_380000_CN402288342/LConn2 -- T_93038661_380000_Pieve_Albignola/LConn2 -- _CN_93038661_380000_CN_62326314_380000/RConn2 -- Pieve_Albignola_Voghera_CN_93038661_380000_CN_98901130_380000/LConn2
  _CN_93038661_380000_CN402288342/LConn3 -- T_93038661_380000_Pieve_Albignola/LConn3 -- _CN_93038661_380000_CN_62326314_380000/RConn3 -- Pieve_Albignola_Voghera_CN_93038661_380000_CN_98901130_380000/LConn3 -- bus337/LConn1
  _CN_93038661_380000_CN402288342/RConn1 -- G_402288342_Stabilimento_di_Ferrera_Erbognone/RConn1 -- _CN_98900549_380000_CN402288342/LConn1
  _CN_93038661_380000_CN402288342/RConn2 -- G_402288342_Stabilimento_di_Ferrera_Erbognone/RConn2 -- _CN_98900549_380000_CN402288342/LConn2
  _CN_93038661_380000_CN402288342/RConn3 -- G_402288342_Stabilimento_di_Ferrera_Erbognone/RConn3 -- _CN_98900549_380000_CN402288342/LConn3 -- bus338/LConn1
  Pieve_Albignola_Voghera_CN_93038661_380000_CN_98901130_380000/RConn1 -- T_98901130_380000_Voghera/LConn1 -- Voghera_Castelnuovo_CN_98901130_380000_CN_98427149_380000/RConn1
  Pieve_Albignola_Voghera_CN_93038661_380000_CN_98901130_380000/RConn2 -- T_98901130_380000_Voghera/LConn2 -- Voghera_Castelnuovo_CN_98901130_380000_CN_98427149_380000/RConn2
  Pieve_Albignola_Voghera_CN_93038661_380000_CN_98901130_380000/RConn3 -- T_98901130_380000_Voghera/LConn3 -- Voghera_Castelnuovo_CN_98901130_380000_CN_98427149_380000/RConn3 -- bus339/LConn1
  Turbigo_Mercallo_CN_72581705_380000_CN_162828577_380000/RConn1 -- T_162828577_380000_Turbigo/LConn1 -- Rondissone___Turbigo_CN_162828577_380000_CN_74869121_380000/RConn1 -- Turbigo_Ospiate_CN_74210017_380000_CN_162828577_380000/LConn1 -- _CN_162828577_380000_CN_62326314_380000/RConn1
  Turbigo_Mercallo_CN_72581705_380000_CN_162828577_380000/RConn2 -- T_162828577_380000_Turbigo/LConn2 -- Rondissone___Turbigo_CN_162828577_380000_CN_74869121_380000/RConn2 -- Turbigo_Ospiate_CN_74210017_380000_CN_162828577_380000/LConn2 -- _CN_162828577_380000_CN_62326314_380000/RConn2
  Turbigo_Mercallo_CN_72581705_380000_CN_162828577_380000/RConn3 -- T_162828577_380000_Turbigo/LConn3 -- Rondissone___Turbigo_CN_162828577_380000_CN_74869121_380000/RConn3 -- bus340/LConn1 -- Turbigo_Ospiate_CN_74210017_380000_CN_162828577_380000/LConn3 -- _CN_162828577_380000_CN_62326314_380000/RConn3
  Carpi_Fossoli_San_Damaso_CN_208398923_380000_CN_148969091_380000/LConn1 -- T_208398923_380000_Carpi_Fossoli/LConn1 -- Carpi_Fossoli_Caorso_CN_208398923_380000_CN_116517585_380000/LConn1
  Carpi_Fossoli_San_Damaso_CN_208398923_380000_CN_148969091_380000/LConn2 -- T_208398923_380000_Carpi_Fossoli/LConn2 -- Carpi_Fossoli_Caorso_CN_208398923_380000_CN_116517585_380000/LConn2
  Carpi_Fossoli_San_Damaso_CN_208398923_380000_CN_148969091_380000/LConn3 -- T_208398923_380000_Carpi_Fossoli/LConn3 -- Carpi_Fossoli_Caorso_CN_208398923_380000_CN_116517585_380000/LConn3 -- bus341/LConn1
  Carpi_Fossoli_San_Damaso_CN_208398923_380000_CN_148969091_380000/RConn1 -- T_148969091_380000;132000;15000_San_Damaso/LConn1 -- San_Damaso_Martignone_CN_338453112_380000_CN_148969091_380000/LConn1
  Carpi_Fossoli_San_Damaso_CN_208398923_380000_CN_148969091_380000/RConn2 -- T_148969091_380000;132000;15000_San_Damaso/LConn2 -- San_Damaso_Martignone_CN_338453112_380000_CN_148969091_380000/LConn2
  Carpi_Fossoli_San_Damaso_CN_208398923_380000_CN_148969091_380000/RConn3 -- T_148969091_380000;132000;15000_San_Damaso/LConn3 -- San_Damaso_Martignone_CN_338453112_380000_CN_148969091_380000/LConn3 -- bus342/LConn1
  Carpi_Fossoli_Caorso_CN_208398923_380000_CN_116517585_380000/RConn1 -- T_116517585_380000_Caorso/LConn1 -- _CN_116517585_380000_CN_211180338_380000/LConn1
  Carpi_Fossoli_Caorso_CN_208398923_380000_CN_116517585_380000/RConn2 -- T_116517585_380000_Caorso/LConn2 -- _CN_116517585_380000_CN_211180338_380000/LConn2
  Carpi_Fossoli_Caorso_CN_208398923_380000_CN_116517585_380000/RConn3 -- T_116517585_380000_Caorso/LConn3 -- _CN_116517585_380000_CN_211180338_380000/LConn3 -- bus343/LConn1
  Pian_della_Speranza___Roma_Nord_CN_83805453_380000_CN_59219335_380000/RConn1 -- T_83805453_380000_Pian_della_Speranza/LConn1 -- Pian_della_Speranza___Roma_Nord_CN_83805453_380000_CN_58931857_380000/LConn1 -- Pian_della_Speranza___Roma_Nord_CN_83805453_380000_CN_80517630_380000/LConn1 -- Poggio_a_Caiano___Pian_della_Speranza_CN_83805453_380000_CN_41360305_380000/RConn1
  Pian_della_Speranza___Roma_Nord_CN_83805453_380000_CN_59219335_380000/RConn2 -- T_83805453_380000_Pian_della_Speranza/LConn2 -- Pian_della_Speranza___Roma_Nord_CN_83805453_380000_CN_58931857_380000/LConn2 -- Pian_della_Speranza___Roma_Nord_CN_83805453_380000_CN_80517630_380000/LConn2 -- Poggio_a_Caiano___Pian_della_Speranza_CN_83805453_380000_CN_41360305_380000/RConn2
  Pian_della_Speranza___Roma_Nord_CN_83805453_380000_CN_59219335_380000/RConn3 -- T_83805453_380000_Pian_della_Speranza/LConn3 -- Pian_della_Speranza___Roma_Nord_CN_83805453_380000_CN_58931857_380000/LConn3 -- Pian_della_Speranza___Roma_Nord_CN_83805453_380000_CN_80517630_380000/LConn3 -- Poggio_a_Caiano___Pian_della_Speranza_CN_83805453_380000_CN_41360305_380000/RConn3 -- bus344/LConn1
  Pian_della_Speranza___Roma_Nord_CN_83805453_380000_CN_58931857_380000/RConn1 -- T_58931857_380000_Valmontone/LConn1 -- Presenzano_Valmontone_CN_58931857_380000_CN_82921983_380000/LConn1 -- _CN_58931857_380000_CN_76709660_380000/LConn1 -- Valmontone_Latina_CN_58931857_380000_CN_339704025_380000/LConn1
  Pian_della_Speranza___Roma_Nord_CN_83805453_380000_CN_58931857_380000/RConn2 -- T_58931857_380000_Valmontone/LConn2 -- Presenzano_Valmontone_CN_58931857_380000_CN_82921983_380000/LConn2 -- _CN_58931857_380000_CN_76709660_380000/LConn2 -- Valmontone_Latina_CN_58931857_380000_CN_339704025_380000/LConn2
  Pian_della_Speranza___Roma_Nord_CN_83805453_380000_CN_58931857_380000/RConn3 -- T_58931857_380000_Valmontone/LConn3 -- Presenzano_Valmontone_CN_58931857_380000_CN_82921983_380000/LConn3 -- _CN_58931857_380000_CN_76709660_380000/LConn3 -- Valmontone_Latina_CN_58931857_380000_CN_339704025_380000/LConn3 -- bus345/LConn1
  Pian_della_Speranza___Roma_Nord_CN_83805453_380000_CN_80517630_380000/RConn1 -- T_80517630_380000_Roma_Nord_smistamento_energia_elettrica_TERNA/LConn1 -- _CN_76709660_380000_CN_80517630_380000/LConn1 -- Santa_Lucia_Roma_Nord_CN_82762493_380000_CN_80517630_380000/LConn1
  Pian_della_Speranza___Roma_Nord_CN_83805453_380000_CN_80517630_380000/RConn2 -- T_80517630_380000_Roma_Nord_smistamento_energia_elettrica_TERNA/LConn2 -- _CN_76709660_380000_CN_80517630_380000/LConn2 -- Santa_Lucia_Roma_Nord_CN_82762493_380000_CN_80517630_380000/LConn2
  Pian_della_Speranza___Roma_Nord_CN_83805453_380000_CN_80517630_380000/RConn3 -- T_80517630_380000_Roma_Nord_smistamento_energia_elettrica_TERNA/LConn3 -- _CN_76709660_380000_CN_80517630_380000/LConn3 -- bus346/LConn1 -- Santa_Lucia_Roma_Nord_CN_82762493_380000_CN_80517630_380000/LConn3
  Dolo___Venezia_Nord_CN_84301904_380000_CN_59153311_380000/LConn1 -- T_84301904_380000_Venezia_Nord/LConn1 -- _CN_84301904_380000_CN_59026315_380000/RConn1
  Dolo___Venezia_Nord_CN_84301904_380000_CN_59153311_380000/LConn2 -- T_84301904_380000_Venezia_Nord/LConn2 -- _CN_84301904_380000_CN_59026315_380000/RConn2
  Dolo___Venezia_Nord_CN_84301904_380000_CN_59153311_380000/LConn3 -- T_84301904_380000_Venezia_Nord/LConn3 -- _CN_84301904_380000_CN_59026315_380000/RConn3 -- bus347/LConn1
  Dolo___Venezia_Nord_CN_84301904_380000_CN_59153311_380000/RConn1 -- T_59153311_380000_Dolo/LConn1 -- _CN_59153311_380000_CN244931645/LConn1 -- _CN_59366523_380000_CN_59153311_380000/LConn1 -- _CN_81929591_380000_CN_59153311_380000/LConn1
  Dolo___Venezia_Nord_CN_84301904_380000_CN_59153311_380000/RConn2 -- T_59153311_380000_Dolo/LConn2 -- _CN_59153311_380000_CN244931645/LConn2 -- _CN_59366523_380000_CN_59153311_380000/LConn2 -- _CN_81929591_380000_CN_59153311_380000/LConn2
  Dolo___Venezia_Nord_CN_84301904_380000_CN_59153311_380000/RConn3 -- T_59153311_380000_Dolo/LConn3 -- _CN_59153311_380000_CN244931645/LConn3 -- bus348/LConn1 -- _CN_59366523_380000_CN_59153311_380000/LConn3 -- _CN_81929591_380000_CN_59153311_380000/LConn3
  Magisano_Scandale_CN_199676823_380000_CN_109756016_380000/RConn1 -- T_109756016_380000_Scandale/LConn1 -- Rossano_Scandale_CN_109756016_380000_CN_109588422_380000/LConn1
  Magisano_Scandale_CN_199676823_380000_CN_109756016_380000/RConn2 -- T_109756016_380000_Scandale/LConn2 -- Rossano_Scandale_CN_109756016_380000_CN_109588422_380000/LConn2
  Magisano_Scandale_CN_199676823_380000_CN_109756016_380000/RConn3 -- T_109756016_380000_Scandale/LConn3 -- Rossano_Scandale_CN_109756016_380000_CN_109588422_380000/LConn3 -- bus349/LConn1
  T_418902799_380000_Brindisi_Sud_centrale_GR_1/LConn1 -- _CN_418902799_380000_CN_60888331_380000/LConn1
  T_418902799_380000_Brindisi_Sud_centrale_GR_1/LConn2 -- _CN_418902799_380000_CN_60888331_380000/LConn2
  _CN_418902799_380000_CN_60888331_380000/LConn3 -- T_418902799_380000_Brindisi_Sud_centrale_GR_1/LConn3 -- bus350/LConn1
  _CN_418902799_380000_CN_60888331_380000/RConn1 -- T_60888331_380000_Brindisi_Sud/LConn1 -- _CN_60888331_380000_CN61814451/LConn1 -- Brindisi_Sud_Matera_CN_103306951_380000_CN_60888331_380000/LConn1 -- _CN_60888331_380000_CN_60919237_380000/RConn1 -- Galatina_Brindisi_sud_CN_60888331_380000_CN_103386958_380000/RConn1 -- Andria_Brindisi_sud_CN_60888331_380000_CN_126203383_380000/LConn1
  _CN_418902799_380000_CN_60888331_380000/RConn2 -- T_60888331_380000_Brindisi_Sud/LConn2 -- _CN_60888331_380000_CN61814451/LConn2 -- Brindisi_Sud_Matera_CN_103306951_380000_CN_60888331_380000/LConn2 -- _CN_60888331_380000_CN_60919237_380000/RConn2 -- Galatina_Brindisi_sud_CN_60888331_380000_CN_103386958_380000/RConn2 -- Andria_Brindisi_sud_CN_60888331_380000_CN_126203383_380000/LConn2
  _CN_418902799_380000_CN_60888331_380000/RConn3 -- T_60888331_380000_Brindisi_Sud/LConn3 -- _CN_60888331_380000_CN61814451/LConn3 -- bus351/LConn1 -- Brindisi_Sud_Matera_CN_103306951_380000_CN_60888331_380000/LConn3 -- _CN_60888331_380000_CN_60919237_380000/RConn3 -- Galatina_Brindisi_sud_CN_60888331_380000_CN_103386958_380000/RConn3 -- Andria_Brindisi_sud_CN_60888331_380000_CN_126203383_380000/LConn3
  _CN_139975773_380000_CN_140710344_380000/RConn1 -- T_140710344_380000_Tavarnuzze/LConn1 -- _CN_140710344_380000_CN_140715391_380000/LConn1
  _CN_139975773_380000_CN_140710344_380000/RConn2 -- T_140710344_380000_Tavarnuzze/LConn2 -- _CN_140710344_380000_CN_140715391_380000/LConn2
  _CN_139975773_380000_CN_140710344_380000/RConn3 -- T_140710344_380000_Tavarnuzze/LConn3 -- _CN_140710344_380000_CN_140715391_380000/LConn3 -- bus352/LConn1
  Focomorto_Ferrara_Nord_CN_363469921_380000_CN_82084013_380000/RConn1 -- T_363469921_380000_Stazione_elettrica_di_Focomorto/LConn1 -- Focomorto_Ravenna_Canala_CN_363469921_380000_CN_81938081_380000/RConn1
  Focomorto_Ferrara_Nord_CN_363469921_380000_CN_82084013_380000/RConn2 -- T_363469921_380000_Stazione_elettrica_di_Focomorto/LConn2 -- Focomorto_Ravenna_Canala_CN_363469921_380000_CN_81938081_380000/RConn2
  Focomorto_Ferrara_Nord_CN_363469921_380000_CN_82084013_380000/RConn3 -- T_363469921_380000_Stazione_elettrica_di_Focomorto/LConn3 -- Focomorto_Ravenna_Canala_CN_363469921_380000_CN_81938081_380000/RConn3 -- bus353/LConn1
  Vignole_La_Spezia_CN_105757794_380000_CN_100952845_380000/RConn1 -- T_100952845_380000_Vignole/LConn1 -- Vignole___Vado_Termica_CN_103653592_380000_CN_100952845_380000/LConn1 -- Vignole_Castelnuovo_CN_100952845_380000_CN_98427149_380000/RConn1
  Vignole_La_Spezia_CN_105757794_380000_CN_100952845_380000/RConn2 -- T_100952845_380000_Vignole/LConn2 -- Vignole___Vado_Termica_CN_103653592_380000_CN_100952845_380000/LConn2 -- Vignole_Castelnuovo_CN_100952845_380000_CN_98427149_380000/RConn2
  Vignole_La_Spezia_CN_105757794_380000_CN_100952845_380000/RConn3 -- T_100952845_380000_Vignole/LConn3 -- Vignole___Vado_Termica_CN_103653592_380000_CN_100952845_380000/LConn3 -- Vignole_Castelnuovo_CN_100952845_380000_CN_98427149_380000/RConn3 -- bus354/LConn1
  G_116176063_Centrale_termoelettrica/RConn1 -- _CN_105757794_380000_CN116176063/RConn1
  G_116176063_Centrale_termoelettrica/RConn2 -- _CN_105757794_380000_CN116176063/RConn2
  _CN_105757794_380000_CN116176063/RConn3 -- G_116176063_Centrale_termoelettrica/RConn3 -- bus355/LConn1
  Planais___Udine_Ovest_CN_58992998_380000_CN_59462263_380000/RConn1 -- T_59462263_380000_Udine_Ovest/LConn1 -- Udine_Ovest___Cordignano_CN_59462263_380000_CN_82083756_380000/LConn1
  Planais___Udine_Ovest_CN_58992998_380000_CN_59462263_380000/RConn2 -- T_59462263_380000_Udine_Ovest/LConn2 -- Udine_Ovest___Cordignano_CN_59462263_380000_CN_82083756_380000/LConn2
  Planais___Udine_Ovest_CN_58992998_380000_CN_59462263_380000/RConn3 -- T_59462263_380000_Udine_Ovest/LConn3 -- Udine_Ovest___Cordignano_CN_59462263_380000_CN_82083756_380000/LConn3 -- bus356/LConn1
  Cagno_Cislago_CN_72570474_380000_CN_75378894_380000/RConn1 -- T_75378894_380000_Cislago/LConn1 -- Bovisio_Cislago_CN_75378894_380000_CN_74677138_380000/RConn1
  Cagno_Cislago_CN_72570474_380000_CN_75378894_380000/RConn2 -- T_75378894_380000_Cislago/LConn2 -- Bovisio_Cislago_CN_75378894_380000_CN_74677138_380000/RConn2
  Cagno_Cislago_CN_72570474_380000_CN_75378894_380000/RConn3 -- T_75378894_380000_Cislago/LConn3 -- Bovisio_Cislago_CN_75378894_380000_CN_74677138_380000/RConn3 -- bus357/LConn1
  Rossano_Scandale_CN_109756016_380000_CN_109588422_380000/RConn1 -- T_109588422_380000_Rossano_Termica/LConn1 -- _CN_108020416_380000_CN_109588422_380000/RConn1
  Rossano_Scandale_CN_109756016_380000_CN_109588422_380000/RConn2 -- T_109588422_380000_Rossano_Termica/LConn2 -- _CN_108020416_380000_CN_109588422_380000/RConn2
  Rossano_Scandale_CN_109756016_380000_CN_109588422_380000/RConn3 -- T_109588422_380000_Rossano_Termica/LConn3 -- _CN_108020416_380000_CN_109588422_380000/RConn3 -- bus358/LConn1
  T_105141365_380000_Laboratori_Cesi_Chivasso/LConn1 -- _CN_105141365_380000_CN_74869121_380000/RConn1
  T_105141365_380000_Laboratori_Cesi_Chivasso/LConn2 -- _CN_105141365_380000_CN_74869121_380000/RConn2
  _CN_105141365_380000_CN_74869121_380000/RConn3 -- T_105141365_380000_Laboratori_Cesi_Chivasso/LConn3 -- bus359/LConn1
  Udine_Ovest___Cordignano_CN_59462263_380000_CN_82083756_380000/RConn1 -- T_82083756_380000_Cordignano/LConn1 -- _CN_64942789_380000_CN_82083756_380000/LConn1
  Udine_Ovest___Cordignano_CN_59462263_380000_CN_82083756_380000/RConn2 -- T_82083756_380000_Cordignano/LConn2 -- _CN_64942789_380000_CN_82083756_380000/LConn2
  Udine_Ovest___Cordignano_CN_59462263_380000_CN_82083756_380000/RConn3 -- T_82083756_380000_Cordignano/LConn3 -- _CN_64942789_380000_CN_82083756_380000/LConn3 -- bus360/LConn1
  Martignone___Sermide_CN_338453112_380000_CN_81931074_380000/LConn1 -- T_338453112_380000_Martignone/LConn1 -- San_Damaso_Martignone_CN_338453112_380000_CN_78066534_380000/RConn1 -- San_Damaso_Martignone_CN_338453112_380000_CN_148969091_380000/RConn1 -- Martignone___Sermide_CN_338453112_380000_CN_139442467_380000/LConn1 -- Martignone___Sermide_CN_338453112_380000_CN_82084019_380000/RConn1 -- Martignone_Bargi_CN_338453112_380000_CN_114931087_380000/RConn1
  Martignone___Sermide_CN_338453112_380000_CN_81931074_380000/LConn2 -- T_338453112_380000_Martignone/LConn2 -- San_Damaso_Martignone_CN_338453112_380000_CN_78066534_380000/RConn2 -- San_Damaso_Martignone_CN_338453112_380000_CN_148969091_380000/RConn2 -- Martignone___Sermide_CN_338453112_380000_CN_139442467_380000/LConn2 -- Martignone___Sermide_CN_338453112_380000_CN_82084019_380000/RConn2 -- Martignone_Bargi_CN_338453112_380000_CN_114931087_380000/RConn2
  Martignone___Sermide_CN_338453112_380000_CN_81931074_380000/LConn3 -- T_338453112_380000_Martignone/LConn3 -- San_Damaso_Martignone_CN_338453112_380000_CN_78066534_380000/RConn3 -- San_Damaso_Martignone_CN_338453112_380000_CN_148969091_380000/RConn3 -- bus361/LConn1 -- Martignone___Sermide_CN_338453112_380000_CN_139442467_380000/LConn3 -- Martignone___Sermide_CN_338453112_380000_CN_82084019_380000/RConn3 -- Martignone_Bargi_CN_338453112_380000_CN_114931087_380000/RConn3
  Martignone___Sermide_CN_338453112_380000_CN_81931074_380000/RConn1 -- T_81931074_380000_Forlì_via_Oraziana/LConn1 -- Linea_352_CN_143585004_380000_CN_81931074_380000/LConn1 -- Porto_Tolle_Ravenna_Canala_CN_81938081_380000_CN_81931074_380000/RConn1
  Martignone___Sermide_CN_338453112_380000_CN_81931074_380000/RConn2 -- T_81931074_380000_Forlì_via_Oraziana/LConn2 -- Linea_352_CN_143585004_380000_CN_81931074_380000/LConn2 -- Porto_Tolle_Ravenna_Canala_CN_81938081_380000_CN_81931074_380000/RConn2
  Martignone___Sermide_CN_338453112_380000_CN_81931074_380000/RConn3 -- T_81931074_380000_Forlì_via_Oraziana/LConn3 -- Linea_352_CN_143585004_380000_CN_81931074_380000/LConn3 -- bus362/LConn1 -- Porto_Tolle_Ravenna_Canala_CN_81938081_380000_CN_81931074_380000/RConn3
  T_139442467_380000_Colunga/LConn1 -- Martignone___Sermide_CN_338453112_380000_CN_139442467_380000/RConn1
  T_139442467_380000_Colunga/LConn2 -- Martignone___Sermide_CN_338453112_380000_CN_139442467_380000/RConn2
  Martignone___Sermide_CN_338453112_380000_CN_139442467_380000/RConn3 -- T_139442467_380000_Colunga/LConn3 -- bus363/LConn1
  _CN_59366523_380000_CN_59153311_380000/RConn1 -- T_59366523_380000;220000;132000_Stazione_elettrica_di_Camin/LConn1 -- _CN_59366523_380000_CN_59556712_380000/RConn1 -- Camin_RFX_CN_59366523_380000_CN_95840602_380000/LConn1
  _CN_59366523_380000_CN_59153311_380000/RConn2 -- T_59366523_380000;220000;132000_Stazione_elettrica_di_Camin/LConn2 -- _CN_59366523_380000_CN_59556712_380000/RConn2 -- Camin_RFX_CN_59366523_380000_CN_95840602_380000/LConn2
  _CN_59366523_380000_CN_59153311_380000/RConn3 -- T_59366523_380000;220000;132000_Stazione_elettrica_di_Camin/LConn3 -- _CN_59366523_380000_CN_59556712_380000/RConn3 -- Camin_RFX_CN_59366523_380000_CN_95840602_380000/LConn3 -- bus364/LConn1
  T_95840602_380000_RFX/LConn1 -- Camin_RFX_CN_59366523_380000_CN_95840602_380000/RConn1
  T_95840602_380000_RFX/LConn2 -- Camin_RFX_CN_59366523_380000_CN_95840602_380000/RConn2
  Camin_RFX_CN_59366523_380000_CN_95840602_380000/RConn3 -- T_95840602_380000_RFX/LConn3 -- bus365/LConn1
  T_146652797_380000_/LConn1 -- _CN_146652797_380000_CN_93860115_380000/LConn1
  T_146652797_380000_/LConn2 -- _CN_146652797_380000_CN_93860115_380000/LConn2
  _CN_146652797_380000_CN_93860115_380000/LConn3 -- T_146652797_380000_/LConn3 -- bus366/LConn1
  _CN_146652797_380000_CN_93860115_380000/RConn1 -- T_93860115_380000_Santa_Maria_Capua_Vetere/LConn1 -- _CN_93860115_380000_CN_84696559_380000/RConn1 -- Sparanise_Santa_Maria_Capua_Vetere_CN_93860115_380000_CN_132450233_380000/LConn1
  _CN_146652797_380000_CN_93860115_380000/RConn2 -- T_93860115_380000_Santa_Maria_Capua_Vetere/LConn2 -- _CN_93860115_380000_CN_84696559_380000/RConn2 -- Sparanise_Santa_Maria_Capua_Vetere_CN_93860115_380000_CN_132450233_380000/LConn2
  _CN_146652797_380000_CN_93860115_380000/RConn3 -- T_93860115_380000_Santa_Maria_Capua_Vetere/LConn3 -- _CN_93860115_380000_CN_84696559_380000/RConn3 -- bus367/LConn1 -- Sparanise_Santa_Maria_Capua_Vetere_CN_93860115_380000_CN_132450233_380000/LConn3
  T_152597636_380000_Bulciago/LConn1 -- _CN_152597636_380000_CN_74677138_380000/RConn1
  T_152597636_380000_Bulciago/LConn2 -- _CN_152597636_380000_CN_74677138_380000/RConn2
  _CN_152597636_380000_CN_74677138_380000/RConn3 -- T_152597636_380000_Bulciago/LConn3 -- bus368/LConn1
  _CN_61375111_380000_CN_60616350_380000/RConn1 -- T_60616350_380000_Gissi_Centrale/LConn1 -- Gissi_Larino_CN_60616350_380000_CN_60235685_380000/RConn1
  _CN_61375111_380000_CN_60616350_380000/RConn2 -- T_60616350_380000_Gissi_Centrale/LConn2 -- Gissi_Larino_CN_60616350_380000_CN_60235685_380000/RConn2
  _CN_61375111_380000_CN_60616350_380000/RConn3 -- T_60616350_380000_Gissi_Centrale/LConn3 -- Gissi_Larino_CN_60616350_380000_CN_60235685_380000/RConn3 -- bus369/LConn1
  T_411026199_380000_ENM_Termoli/LConn1 -- _CN_411026199_380000_CN_60235685_380000/RConn1
  T_411026199_380000_ENM_Termoli/LConn2 -- _CN_411026199_380000_CN_60235685_380000/RConn2
  _CN_411026199_380000_CN_60235685_380000/RConn3 -- T_411026199_380000_ENM_Termoli/LConn3 -- bus370/LConn1
  T_131291789_380000_Lonato/LConn1 -- Lonato_Nogarole_Rocca_CN_131291789_380000_CN_155791516_380000/LConn1
  T_131291789_380000_Lonato/LConn2 -- Lonato_Nogarole_Rocca_CN_131291789_380000_CN_155791516_380000/LConn2
  Lonato_Nogarole_Rocca_CN_131291789_380000_CN_155791516_380000/LConn3 -- T_131291789_380000_Lonato/LConn3 -- bus371/LConn1
  Lonato_Nogarole_Rocca_CN_131291789_380000_CN_155791516_380000/RConn1 -- T_155791516_380000_Nogarole_Rocca/LConn1 -- Dugale_Nogarole_Rocca_CN_155791516_380000_CN_59556712_380000/RConn1
  Lonato_Nogarole_Rocca_CN_131291789_380000_CN_155791516_380000/RConn2 -- T_155791516_380000_Nogarole_Rocca/LConn2 -- Dugale_Nogarole_Rocca_CN_155791516_380000_CN_59556712_380000/RConn2
  Lonato_Nogarole_Rocca_CN_131291789_380000_CN_155791516_380000/RConn3 -- T_155791516_380000_Nogarole_Rocca/LConn3 -- Dugale_Nogarole_Rocca_CN_155791516_380000_CN_59556712_380000/RConn3 -- bus372/LConn1
  T_209982720_380000_Troia/LConn1 -- _CN_418565263_380000_CN_209982720_380000/RConn1
  T_209982720_380000_Troia/LConn2 -- _CN_418565263_380000_CN_209982720_380000/RConn2
  _CN_418565263_380000_CN_209982720_380000/RConn3 -- T_209982720_380000_Troia/LConn3 -- bus373/LConn1
  _CN_418565263_380000_CN_338795626_380000/RConn1 -- T_338795626_380000_Deliceto/LConn1 -- Candela_Deliceto_CN_171270810_380000_CN_338795626_380000/LConn1
  _CN_418565263_380000_CN_338795626_380000/RConn2 -- T_338795626_380000_Deliceto/LConn2 -- Candela_Deliceto_CN_171270810_380000_CN_338795626_380000/LConn2
  _CN_418565263_380000_CN_338795626_380000/RConn3 -- T_338795626_380000_Deliceto/LConn3 -- Candela_Deliceto_CN_171270810_380000_CN_338795626_380000/LConn3 -- bus374/LConn1
  Andria_Foggia_CN_418565263_380000_CN_126203383_380000/RConn1 -- T_126203383_380000_Andria/LConn1 -- Andria_Brindisi_sud_CN_60888331_380000_CN_126203383_380000/RConn1
  Andria_Foggia_CN_418565263_380000_CN_126203383_380000/RConn2 -- T_126203383_380000_Andria/LConn2 -- Andria_Brindisi_sud_CN_60888331_380000_CN_126203383_380000/RConn2
  Andria_Foggia_CN_418565263_380000_CN_126203383_380000/RConn3 -- T_126203383_380000_Andria/LConn3 -- Andria_Brindisi_sud_CN_60888331_380000_CN_126203383_380000/RConn3 -- bus375/LConn1
  Presenzano_Valmontone_CN_58931857_380000_CN_82921983_380000/RConn1 -- T_82921983_380000_Presenzano/LConn1 -- Presenzano_Garigliano_CN_83872215_380000_CN_82921983_380000/LConn1 -- _CN_83058212_380000_CN_82921983_380000/LConn1
  Presenzano_Valmontone_CN_58931857_380000_CN_82921983_380000/RConn2 -- T_82921983_380000_Presenzano/LConn2 -- Presenzano_Garigliano_CN_83872215_380000_CN_82921983_380000/LConn2 -- _CN_83058212_380000_CN_82921983_380000/LConn2
  Presenzano_Valmontone_CN_58931857_380000_CN_82921983_380000/RConn3 -- T_82921983_380000_Presenzano/LConn3 -- Presenzano_Garigliano_CN_83872215_380000_CN_82921983_380000/LConn3 -- bus376/LConn1 -- _CN_83058212_380000_CN_82921983_380000/LConn3
  _CN_58931857_380000_CN_76709660_380000/RConn1 -- T_76709660_380000_Roma_Est/LConn1 -- _CN_76709660_380000_CN_80517630_380000/RConn1
  _CN_58931857_380000_CN_76709660_380000/RConn2 -- T_76709660_380000_Roma_Est/LConn2 -- _CN_76709660_380000_CN_80517630_380000/RConn2
  _CN_58931857_380000_CN_76709660_380000/RConn3 -- T_76709660_380000_Roma_Est/LConn3 -- _CN_76709660_380000_CN_80517630_380000/RConn3 -- bus377/LConn1
  Valmontone_Latina_CN_58931857_380000_CN_339704025_380000/RConn1 -- T_339704025_380000_Latina/LConn1 -- Latina_Ceprano_CN_339704025_380000_CN61012012/LConn1 -- Garigliano_Latina_CN_339704025_380000_CN_83872215_380000/LConn1 -- Latina_Aprilia_380_CN_339704025_380000_CN_172302572_380000/LConn1 -- _CN_76705565_380000_CN_339704025_380000/LConn1
  Valmontone_Latina_CN_58931857_380000_CN_339704025_380000/RConn2 -- T_339704025_380000_Latina/LConn2 -- Latina_Ceprano_CN_339704025_380000_CN61012012/LConn2 -- Garigliano_Latina_CN_339704025_380000_CN_83872215_380000/LConn2 -- Latina_Aprilia_380_CN_339704025_380000_CN_172302572_380000/LConn2 -- _CN_76705565_380000_CN_339704025_380000/LConn2
  Valmontone_Latina_CN_58931857_380000_CN_339704025_380000/RConn3 -- T_339704025_380000_Latina/LConn3 -- Latina_Ceprano_CN_339704025_380000_CN61012012/LConn3 -- Garigliano_Latina_CN_339704025_380000_CN_83872215_380000/LConn3 -- Latina_Aprilia_380_CN_339704025_380000_CN_172302572_380000/LConn3 -- bus378/LConn1 -- _CN_76705565_380000_CN_339704025_380000/LConn3
  T_104359058_380000_Entracque/LConn1 -- Entracque_Magliano_1_CN_104359058_380000_CN_99694910_380000/LConn1
  T_104359058_380000_Entracque/LConn2 -- Entracque_Magliano_1_CN_104359058_380000_CN_99694910_380000/LConn2
  Entracque_Magliano_1_CN_104359058_380000_CN_99694910_380000/LConn3 -- T_104359058_380000_Entracque/LConn3 -- bus379/LConn1
  Entracque_Magliano_1_CN_104359058_380000_CN_99694910_380000/RConn1 -- T_99694910_380000_Magliano/LConn1 -- Magliano_Vado_Termica_CN_103653592_380000_CN_99694910_380000/LConn1 -- Casanova___Magliano_CN_99694910_380000_CN_99826025_380000/LConn1 -- Magliano_Piossasco_CN_99694910_380000_CN_98902899_380000/LConn1
  Entracque_Magliano_1_CN_104359058_380000_CN_99694910_380000/RConn2 -- T_99694910_380000_Magliano/LConn2 -- Magliano_Vado_Termica_CN_103653592_380000_CN_99694910_380000/LConn2 -- Casanova___Magliano_CN_99694910_380000_CN_99826025_380000/LConn2 -- Magliano_Piossasco_CN_99694910_380000_CN_98902899_380000/LConn2
  Entracque_Magliano_1_CN_104359058_380000_CN_99694910_380000/RConn3 -- T_99694910_380000_Magliano/LConn3 -- Magliano_Vado_Termica_CN_103653592_380000_CN_99694910_380000/LConn3 -- Casanova___Magliano_CN_99694910_380000_CN_99826025_380000/LConn3 -- Magliano_Piossasco_CN_99694910_380000_CN_98902899_380000/LConn3 -- bus380/LConn1
  Priolo_Chiaramonte_Gulfi_CN_338753171_380000_CN_57384507_380000/LConn1 -- T_338753171_380000_Priolo/LConn1 -- Priolo_PC_Isab_CN_338753171_380000_CN_415431845_380000/LConn1
  Priolo_Chiaramonte_Gulfi_CN_338753171_380000_CN_57384507_380000/LConn2 -- T_338753171_380000_Priolo/LConn2 -- Priolo_PC_Isab_CN_338753171_380000_CN_415431845_380000/LConn2
  Priolo_Chiaramonte_Gulfi_CN_338753171_380000_CN_57384507_380000/LConn3 -- T_338753171_380000_Priolo/LConn3 -- Priolo_PC_Isab_CN_338753171_380000_CN_415431845_380000/LConn3 -- bus381/LConn1
  Priolo_Chiaramonte_Gulfi_CN_338753171_380000_CN_57384507_380000/RConn1 -- T_57384507_380000_Chiaramonte_Gulfi/LConn1 -- Paternò_Chiaramonte_Gulfi_CN_57384507_380000_CN_61157826_380000/LConn1
  Priolo_Chiaramonte_Gulfi_CN_338753171_380000_CN_57384507_380000/RConn2 -- T_57384507_380000_Chiaramonte_Gulfi/LConn2 -- Paternò_Chiaramonte_Gulfi_CN_57384507_380000_CN_61157826_380000/LConn2
  Priolo_Chiaramonte_Gulfi_CN_338753171_380000_CN_57384507_380000/RConn3 -- T_57384507_380000_Chiaramonte_Gulfi/LConn3 -- Paternò_Chiaramonte_Gulfi_CN_57384507_380000_CN_61157826_380000/LConn3 -- bus382/LConn1
  T_415431845_380000_Isab_Energy/LConn1 -- Priolo_PC_Isab_CN_338753171_380000_CN_415431845_380000/RConn1
  T_415431845_380000_Isab_Energy/LConn2 -- Priolo_PC_Isab_CN_338753171_380000_CN_415431845_380000/RConn2
  Priolo_PC_Isab_CN_338753171_380000_CN_415431845_380000/RConn3 -- T_415431845_380000_Isab_Energy/LConn3 -- bus383/LConn1
  T_146791215__/LConn1 -- _CN_146791061_380000_CN_146791215_380000/RConn1
  T_146791215__/LConn2 -- _CN_146791061_380000_CN_146791215_380000/RConn2
  _CN_146791061_380000_CN_146791215_380000/RConn3 -- T_146791215__/LConn3 -- bus384/LConn1
  T_171270810_380000_Candela/LConn1 -- Candela_Deliceto_CN_171270810_380000_CN_338795626_380000/RConn1
  T_171270810_380000_Candela/LConn2 -- Candela_Deliceto_CN_171270810_380000_CN_338795626_380000/RConn2
  Candela_Deliceto_CN_171270810_380000_CN_338795626_380000/RConn3 -- T_171270810_380000_Candela/LConn3 -- bus385/LConn1
  Porto_Tolle_Ravenna_Canala_CN_81938081_380000_CN_81929591_380000/RConn1 -- T_81929591_380000_Porto_Tolle/LConn1 -- _CN_81929591_380000_CN_155158689_380000/LConn1 -- _CN_81929591_380000_CN_59153311_380000/RConn1 -- _CN_81929591_380000_CN81944353/LConn1
  Porto_Tolle_Ravenna_Canala_CN_81938081_380000_CN_81929591_380000/RConn2 -- T_81929591_380000_Porto_Tolle/LConn2 -- _CN_81929591_380000_CN_155158689_380000/LConn2 -- _CN_81929591_380000_CN_59153311_380000/RConn2 -- _CN_81929591_380000_CN81944353/LConn2
  Porto_Tolle_Ravenna_Canala_CN_81938081_380000_CN_81929591_380000/RConn3 -- T_81929591_380000_Porto_Tolle/LConn3 -- _CN_81929591_380000_CN_155158689_380000/LConn3 -- _CN_81929591_380000_CN_59153311_380000/RConn3 -- bus386/LConn1 -- _CN_81929591_380000_CN81944353/LConn3
  T_158739183_380000_Porto_Corsini_Sezione_1/LConn1 -- Centrale_Teodora___Ravenna_Canala_CN_81938081_380000_CN_158739183_380000/RConn1
  T_158739183_380000_Porto_Corsini_Sezione_1/LConn2 -- Centrale_Teodora___Ravenna_Canala_CN_81938081_380000_CN_158739183_380000/RConn2
  Centrale_Teodora___Ravenna_Canala_CN_81938081_380000_CN_158739183_380000/RConn3 -- T_158739183_380000_Porto_Corsini_Sezione_1/LConn3 -- bus387/LConn1
  T_64200868_380000_Stazione_Primaria_di_Edolo/LConn1 -- _CN_64200868_380000_CN_72466334_380000/LConn1
  T_64200868_380000_Stazione_Primaria_di_Edolo/LConn2 -- _CN_64200868_380000_CN_72466334_380000/LConn2
  _CN_64200868_380000_CN_72466334_380000/LConn3 -- T_64200868_380000_Stazione_Primaria_di_Edolo/LConn3 -- bus388/LConn1
  _CN_64200868_380000_CN_72466334_380000/RConn1 -- T_72466334_380000_San_Fiorano/LConn1 -- _CN_72466334_380000_CN_75602396_380000/LConn1 -- _CN_72466334_380000_CN_42206116_380000/LConn1
  _CN_64200868_380000_CN_72466334_380000/RConn2 -- T_72466334_380000_San_Fiorano/LConn2 -- _CN_72466334_380000_CN_75602396_380000/LConn2 -- _CN_72466334_380000_CN_42206116_380000/LConn2
  _CN_64200868_380000_CN_72466334_380000/RConn3 -- T_72466334_380000_San_Fiorano/LConn3 -- _CN_72466334_380000_CN_75602396_380000/LConn3 -- _CN_72466334_380000_CN_42206116_380000/LConn3 -- bus389/LConn1
  T_365525159_380000_SEF_Ferrara/LConn1 -- _CN_365525159_380000_CN_82084013_380000/RConn1
  T_365525159_380000_SEF_Ferrara/LConn2 -- _CN_365525159_380000_CN_82084013_380000/RConn2
  _CN_365525159_380000_CN_82084013_380000/RConn3 -- T_365525159_380000_SEF_Ferrara/LConn3 -- bus390/LConn1
  G_281858231_Centrale_Rizziconi/RConn1 -- _CN_109993642_380000_CN281858231/RConn1
  G_281858231_Centrale_Rizziconi/RConn2 -- _CN_109993642_380000_CN281858231/RConn2
  _CN_109993642_380000_CN281858231/RConn3 -- G_281858231_Centrale_Rizziconi/RConn3 -- bus391/LConn1
  Aliano___Matera_CN_103306951_380000_CN_338790588_380000/LConn1 -- T_103306951_380000_Matera/LConn1 -- Matera_Bisaccia_CN_103306951_380000_CN_257351439_380000/LConn1 -- Brindisi_Sud_Matera_CN_103306951_380000_CN_60888331_380000/RConn1 -- Castellaneta_Matera_CN_103306951_380000_CN_338760116_380000/RConn1
  Aliano___Matera_CN_103306951_380000_CN_338790588_380000/LConn2 -- T_103306951_380000_Matera/LConn2 -- Matera_Bisaccia_CN_103306951_380000_CN_257351439_380000/LConn2 -- Brindisi_Sud_Matera_CN_103306951_380000_CN_60888331_380000/RConn2 -- Castellaneta_Matera_CN_103306951_380000_CN_338760116_380000/RConn2
  Aliano___Matera_CN_103306951_380000_CN_338790588_380000/LConn3 -- T_103306951_380000_Matera/LConn3 -- Matera_Bisaccia_CN_103306951_380000_CN_257351439_380000/LConn3 -- bus392/LConn1 -- Brindisi_Sud_Matera_CN_103306951_380000_CN_60888331_380000/RConn3 -- Castellaneta_Matera_CN_103306951_380000_CN_338760116_380000/RConn3
  Aliano___Matera_CN_103306951_380000_CN_338790588_380000/RConn1 -- T_338790588_380000_Aliano/LConn1 -- _CN_338790588_380000_CN_108020416_380000/RConn1
  Aliano___Matera_CN_103306951_380000_CN_338790588_380000/RConn2 -- T_338790588_380000_Aliano/LConn2 -- _CN_338790588_380000_CN_108020416_380000/RConn2
  Aliano___Matera_CN_103306951_380000_CN_338790588_380000/RConn3 -- T_338790588_380000_Aliano/LConn3 -- _CN_338790588_380000_CN_108020416_380000/RConn3 -- bus393/LConn1
  Matera_Bisaccia_CN_103306951_380000_CN_257351439_380000/RConn1 -- T_257351439_380000_Bisaccia_380/LConn1 -- _CN_257351439_380000_CN_84696559_380000/RConn1
  Matera_Bisaccia_CN_103306951_380000_CN_257351439_380000/RConn2 -- T_257351439_380000_Bisaccia_380/LConn2 -- _CN_257351439_380000_CN_84696559_380000/RConn2
  Matera_Bisaccia_CN_103306951_380000_CN_257351439_380000/RConn3 -- T_257351439_380000_Bisaccia_380/LConn3 -- _CN_257351439_380000_CN_84696559_380000/RConn3 -- bus394/LConn1
  Fiumesanto_Codrongianos_CN_409439916_380000_CN_61743815_380000/LConn1 -- T_409439916_380000_Fiumesanto_Carbo_380/LConn1 -- Ittiri_Fiumesanto_CN_409439916_380000_CN_144005863_380000/LConn1
  Fiumesanto_Codrongianos_CN_409439916_380000_CN_61743815_380000/LConn2 -- T_409439916_380000_Fiumesanto_Carbo_380/LConn2 -- Ittiri_Fiumesanto_CN_409439916_380000_CN_144005863_380000/LConn2
  Fiumesanto_Codrongianos_CN_409439916_380000_CN_61743815_380000/LConn3 -- T_409439916_380000_Fiumesanto_Carbo_380/LConn3 -- Ittiri_Fiumesanto_CN_409439916_380000_CN_144005863_380000/LConn3 -- bus395/LConn1
  Fiumesanto_Codrongianos_CN_409439916_380000_CN_61743815_380000/RConn1 -- T_61743815_380000;220000;150000_Codrongianos/LConn1 -- Ittiri_Codrongianos_CN_61743815_380000_CN_144005863_380000/LConn1
  Fiumesanto_Codrongianos_CN_409439916_380000_CN_61743815_380000/RConn2 -- T_61743815_380000;220000;150000_Codrongianos/LConn2 -- Ittiri_Codrongianos_CN_61743815_380000_CN_144005863_380000/LConn2
  Fiumesanto_Codrongianos_CN_409439916_380000_CN_61743815_380000/RConn3 -- T_61743815_380000;220000;150000_Codrongianos/LConn3 -- Ittiri_Codrongianos_CN_61743815_380000_CN_144005863_380000/LConn3 -- bus396/LConn1
  Ittiri_Fiumesanto_CN_409439916_380000_CN_144005863_380000/RConn1 -- T_144005863_380000_Ittiri/LConn1 -- Ittiri_Codrongianos_CN_61743815_380000_CN_144005863_380000/RConn1 -- Ittiri_Selargius_CN_144005863_380000_CN_118987056_380000/LConn1
  Ittiri_Fiumesanto_CN_409439916_380000_CN_144005863_380000/RConn2 -- T_144005863_380000_Ittiri/LConn2 -- Ittiri_Codrongianos_CN_61743815_380000_CN_144005863_380000/RConn2 -- Ittiri_Selargius_CN_144005863_380000_CN_118987056_380000/LConn2
  Ittiri_Fiumesanto_CN_409439916_380000_CN_144005863_380000/RConn3 -- T_144005863_380000_Ittiri/LConn3 -- Ittiri_Codrongianos_CN_61743815_380000_CN_144005863_380000/RConn3 -- Ittiri_Selargius_CN_144005863_380000_CN_118987056_380000/LConn3 -- bus397/LConn1
  _CN_140710344_380000_CN_140715391_380000/RConn1 -- T_140715391_380000_Le_Rose/LConn1 -- _CN_339703159_380000_CN_140715391_380000/LConn1
  _CN_140710344_380000_CN_140715391_380000/RConn2 -- T_140715391_380000_Le_Rose/LConn2 -- _CN_339703159_380000_CN_140715391_380000/LConn2
  _CN_140710344_380000_CN_140715391_380000/RConn3 -- T_140715391_380000_Le_Rose/LConn3 -- _CN_339703159_380000_CN_140715391_380000/LConn3 -- bus398/LConn1
  Flero_Cremona_CN_58440884_380000_CN_211180338_380000/LConn1 -- T_58440884_380000_Flero/LConn1 -- Flero_Mantova_CN_58440884_380000_CN_116697005_380000/RConn1 -- Flero_Cremona_CN_58440884_380000_CN_116518388_380000/LConn1 -- Flero_Travagliato_CN_58440884_380000_CN_120356593_380000/LConn1
  Flero_Cremona_CN_58440884_380000_CN_211180338_380000/LConn2 -- T_58440884_380000_Flero/LConn2 -- Flero_Mantova_CN_58440884_380000_CN_116697005_380000/RConn2 -- Flero_Cremona_CN_58440884_380000_CN_116518388_380000/LConn2 -- Flero_Travagliato_CN_58440884_380000_CN_120356593_380000/LConn2
  Flero_Cremona_CN_58440884_380000_CN_211180338_380000/LConn3 -- T_58440884_380000_Flero/LConn3 -- Flero_Mantova_CN_58440884_380000_CN_116697005_380000/RConn3 -- bus399/LConn1 -- Flero_Cremona_CN_58440884_380000_CN_116518388_380000/LConn3 -- Flero_Travagliato_CN_58440884_380000_CN_120356593_380000/LConn3
  Flero_Cremona_CN_58440884_380000_CN_211180338_380000/RConn1 -- T_211180338_380000_Maleo/LConn1 -- Maleo_San_Rocco_CN_211180338_380000_CN_93315059_380000/RConn1 -- _CN_211180338_380000_CN_202271565_380000/RConn1 -- _CN_116517585_380000_CN_211180338_380000/RConn1
  Flero_Cremona_CN_58440884_380000_CN_211180338_380000/RConn2 -- T_211180338_380000_Maleo/LConn2 -- Maleo_San_Rocco_CN_211180338_380000_CN_93315059_380000/RConn2 -- _CN_211180338_380000_CN_202271565_380000/RConn2 -- _CN_116517585_380000_CN_211180338_380000/RConn2
  Flero_Cremona_CN_58440884_380000_CN_211180338_380000/RConn3 -- T_211180338_380000_Maleo/LConn3 -- Maleo_San_Rocco_CN_211180338_380000_CN_93315059_380000/RConn3 -- _CN_211180338_380000_CN_202271565_380000/RConn3 -- bus400/LConn1 -- _CN_116517585_380000_CN_211180338_380000/RConn3
  Flero_Cremona_CN_58440884_380000_CN_116518388_380000/RConn1 -- T_116518388_380000_Cremona/LConn1 -- _CN_116518388_380000_CN_116519166_380000/LConn1
  Flero_Cremona_CN_58440884_380000_CN_116518388_380000/RConn2 -- T_116518388_380000_Cremona/LConn2 -- _CN_116518388_380000_CN_116519166_380000/LConn2
  Flero_Cremona_CN_58440884_380000_CN_116518388_380000/RConn3 -- T_116518388_380000_Cremona/LConn3 -- _CN_116518388_380000_CN_116519166_380000/LConn3 -- bus401/LConn1
  Flero_Travagliato_CN_58440884_380000_CN_120356593_380000/RConn1 -- T_120356593_380000_Travagliato/LConn1 -- Chiari_Travagliato_CN_120356593_380000_CN_72475426_380000/LConn1
  Flero_Travagliato_CN_58440884_380000_CN_120356593_380000/RConn2 -- T_120356593_380000_Travagliato/LConn2 -- Chiari_Travagliato_CN_120356593_380000_CN_72475426_380000/LConn2
  Flero_Travagliato_CN_58440884_380000_CN_120356593_380000/RConn3 -- T_120356593_380000_Travagliato/LConn3 -- Chiari_Travagliato_CN_120356593_380000_CN_72475426_380000/LConn3 -- bus402/LConn1
  _CN_64942789_380000_CN_59556712_380000/RConn1 -- T_64942789_380000;132000_Sandrigo/LConn1 -- _CN_64942789_380000_CN_82083756_380000/RConn1
  _CN_64942789_380000_CN_59556712_380000/RConn2 -- T_64942789_380000;132000_Sandrigo/LConn2 -- _CN_64942789_380000_CN_82083756_380000/RConn2
  _CN_64942789_380000_CN_59556712_380000/RConn3 -- T_64942789_380000;132000_Sandrigo/LConn3 -- _CN_64942789_380000_CN_82083756_380000/RConn3 -- bus403/LConn1
  T_158086858__/LConn1 -- _CN_158086858_380000_CN_158183759_380000/LConn1
  T_158086858__/LConn2 -- _CN_158086858_380000_CN_158183759_380000/LConn2
  _CN_158086858_380000_CN_158183759_380000/LConn3 -- T_158086858__/LConn3 -- bus404/LConn1
  T_158183759__/LConn1 -- _CN_158086858_380000_CN_158183759_380000/RConn1
  T_158183759__/LConn2 -- _CN_158086858_380000_CN_158183759_380000/RConn2
  _CN_158086858_380000_CN_158183759_380000/RConn3 -- T_158183759__/LConn3 -- bus405/LConn1
  T_339703159_380000_Santa_Barbara/LConn1 -- _CN_339703159_380000_CN_140715391_380000/RConn1
  T_339703159_380000_Santa_Barbara/LConn2 -- _CN_339703159_380000_CN_140715391_380000/RConn2
  _CN_339703159_380000_CN_140715391_380000/RConn3 -- T_339703159_380000_Santa_Barbara/LConn3 -- bus406/LConn1
  Garigliano_Patria_CN_114661587_380000_CN_83872215_380000/LConn1 -- T_114661587_380000_Patria/LConn1 -- _CN_114661587_380000_CN_84696559_380000/RConn1
  Garigliano_Patria_CN_114661587_380000_CN_83872215_380000/LConn2 -- T_114661587_380000_Patria/LConn2 -- _CN_114661587_380000_CN_84696559_380000/RConn2
  Garigliano_Patria_CN_114661587_380000_CN_83872215_380000/LConn3 -- T_114661587_380000_Patria/LConn3 -- _CN_114661587_380000_CN_84696559_380000/RConn3 -- bus407/LConn1
  Garigliano_Patria_CN_114661587_380000_CN_83872215_380000/RConn1 -- T_83872215_380000_Garigliano/LConn1 -- Sparanise_Garigliano_CN_132450233_380000_CN_83872215_380000/LConn1 -- Presenzano_Garigliano_CN_83872215_380000_CN_82921983_380000/RConn1 -- Garigliano_Latina_CN_339704025_380000_CN_83872215_380000/RConn1 -- Garigliano_Ceprano_CN_339706878_380000_CN_83872215_380000/LConn1
  Garigliano_Patria_CN_114661587_380000_CN_83872215_380000/RConn2 -- T_83872215_380000_Garigliano/LConn2 -- Sparanise_Garigliano_CN_132450233_380000_CN_83872215_380000/LConn2 -- Presenzano_Garigliano_CN_83872215_380000_CN_82921983_380000/RConn2 -- Garigliano_Latina_CN_339704025_380000_CN_83872215_380000/RConn2 -- Garigliano_Ceprano_CN_339706878_380000_CN_83872215_380000/LConn2
  Garigliano_Patria_CN_114661587_380000_CN_83872215_380000/RConn3 -- T_83872215_380000_Garigliano/LConn3 -- Sparanise_Garigliano_CN_132450233_380000_CN_83872215_380000/LConn3 -- Presenzano_Garigliano_CN_83872215_380000_CN_82921983_380000/RConn3 -- bus408/LConn1 -- Garigliano_Latina_CN_339704025_380000_CN_83872215_380000/RConn3 -- Garigliano_Ceprano_CN_339706878_380000_CN_83872215_380000/LConn3
  _CN_82759380_380000_CN_82762493_380000/LConn1 -- T_82759380_380000_Aurelia/LConn1 -- _CN_82759380_380000_CN_82114903_380000/LConn1 -- _CN_82759380_380000_CN_59219335_380000/RConn1 -- Aurelia_Roma_sud_CN_82759380_380000_CN_76705565_380000/LConn1
  _CN_82759380_380000_CN_82762493_380000/LConn2 -- T_82759380_380000_Aurelia/LConn2 -- _CN_82759380_380000_CN_82114903_380000/LConn2 -- _CN_82759380_380000_CN_59219335_380000/RConn2 -- Aurelia_Roma_sud_CN_82759380_380000_CN_76705565_380000/LConn2
  _CN_82759380_380000_CN_82762493_380000/LConn3 -- T_82759380_380000_Aurelia/LConn3 -- _CN_82759380_380000_CN_82114903_380000/LConn3 -- _CN_82759380_380000_CN_59219335_380000/RConn3 -- bus409/LConn1 -- Aurelia_Roma_sud_CN_82759380_380000_CN_76705565_380000/LConn3
  _CN_82759380_380000_CN_82762493_380000/RConn1 -- T_82762493_380000_Santa_Lucia/LConn1 -- _CN_82762493_380000_CN_82767145_380000/LConn1 -- Santa_Lucia_Roma_Ovest_CN_82762493_380000_CN_80399102_380000/LConn1 -- Santa_Lucia_Roma_Nord_CN_82762493_380000_CN_80517630_380000/RConn1
  _CN_82759380_380000_CN_82762493_380000/RConn2 -- T_82762493_380000_Santa_Lucia/LConn2 -- _CN_82762493_380000_CN_82767145_380000/LConn2 -- Santa_Lucia_Roma_Ovest_CN_82762493_380000_CN_80399102_380000/LConn2 -- Santa_Lucia_Roma_Nord_CN_82762493_380000_CN_80517630_380000/RConn2
  _CN_82759380_380000_CN_82762493_380000/RConn3 -- T_82762493_380000_Santa_Lucia/LConn3 -- _CN_82762493_380000_CN_82767145_380000/LConn3 -- bus410/LConn1 -- Santa_Lucia_Roma_Ovest_CN_82762493_380000_CN_80399102_380000/LConn3 -- Santa_Lucia_Roma_Nord_CN_82762493_380000_CN_80517630_380000/RConn3
  Aurelia_Roma_sud_CN_82759380_380000_CN_76705565_380000/RConn1 -- T_76705565_380000;220000;150000_Roma_Sud/LConn1 -- Roma_Sud_Roma_Ovest_CN_80399102_380000_CN_76705565_380000/LConn1 -- Roma_Sud_Aprilia_380_CN_76705565_380000_CN_172302572_380000/LConn1 -- _CN_76705565_380000_CN_339704025_380000/RConn1
  Aurelia_Roma_sud_CN_82759380_380000_CN_76705565_380000/RConn2 -- T_76705565_380000;220000;150000_Roma_Sud/LConn2 -- Roma_Sud_Roma_Ovest_CN_80399102_380000_CN_76705565_380000/LConn2 -- Roma_Sud_Aprilia_380_CN_76705565_380000_CN_172302572_380000/LConn2 -- _CN_76705565_380000_CN_339704025_380000/RConn2
  Aurelia_Roma_sud_CN_82759380_380000_CN_76705565_380000/RConn3 -- T_76705565_380000;220000;150000_Roma_Sud/LConn3 -- Roma_Sud_Roma_Ovest_CN_80399102_380000_CN_76705565_380000/LConn3 -- Roma_Sud_Aprilia_380_CN_76705565_380000_CN_172302572_380000/LConn3 -- _CN_76705565_380000_CN_339704025_380000/RConn3 -- bus411/LConn1
  T_82114903_380000_Torrevaldiga_Nord/LConn1 -- _CN_82759380_380000_CN_82114903_380000/RConn1
  T_82114903_380000_Torrevaldiga_Nord/LConn2 -- _CN_82759380_380000_CN_82114903_380000/RConn2
  _CN_82759380_380000_CN_82114903_380000/RConn3 -- T_82114903_380000_Torrevaldiga_Nord/LConn3 -- bus412/LConn1
  Vignole___Vado_Termica_CN_103653592_380000_CN_100952845_380000/RConn1 -- T_103653592_380000_Vado_Termica/LConn1 -- Magliano_Vado_Termica_CN_103653592_380000_CN_99694910_380000/RConn1
  Vignole___Vado_Termica_CN_103653592_380000_CN_100952845_380000/RConn2 -- T_103653592_380000_Vado_Termica/LConn2 -- Magliano_Vado_Termica_CN_103653592_380000_CN_99694910_380000/RConn2
  Vignole___Vado_Termica_CN_103653592_380000_CN_100952845_380000/RConn3 -- T_103653592_380000_Vado_Termica/LConn3 -- Magliano_Vado_Termica_CN_103653592_380000_CN_99694910_380000/RConn3 -- bus413/LConn1
  T_83058212_380000_Benevento_2/LConn1 -- _CN_83058212_380000_CN_82921983_380000/RConn1
  T_83058212_380000_Benevento_2/LConn2 -- _CN_83058212_380000_CN_82921983_380000/RConn2
  _CN_83058212_380000_CN_82921983_380000/RConn3 -- T_83058212_380000_Benevento_2/LConn3 -- bus414/LConn1
  T_116797658_380000_Mantova_380/LConn1 -- _CN_116797658_380000_CN_116912085_380000/LConn1
  T_116797658_380000_Mantova_380/LConn2 -- _CN_116797658_380000_CN_116912085_380000/LConn2
  _CN_116797658_380000_CN_116912085_380000/LConn3 -- T_116797658_380000_Mantova_380/LConn3 -- bus415/LConn1
  _CN_116797658_380000_CN_116912085_380000/RConn1 -- T_116912085__/LConn1 -- _CN_116697005_380000_CN_116912085_380000/RConn1
  _CN_116797658_380000_CN_116912085_380000/RConn2 -- T_116912085__/LConn2 -- _CN_116697005_380000_CN_116912085_380000/RConn2
  _CN_116797658_380000_CN_116912085_380000/RConn3 -- T_116912085__/LConn3 -- _CN_116697005_380000_CN_116912085_380000/RConn3 -- bus416/LConn1
  T_255011550_380000_Sarlux/LConn1 -- _CN_255011550_380000_CN_255011551_380000/LConn1
  T_255011550_380000_Sarlux/LConn2 -- _CN_255011550_380000_CN_255011551_380000/LConn2
  _CN_255011550_380000_CN_255011551_380000/LConn3 -- T_255011550_380000_Sarlux/LConn3 -- bus417/LConn1
  T_255011551_380000_Cagliari_Sud/LConn1 -- _CN_255011550_380000_CN_255011551_380000/RConn1
  T_255011551_380000_Cagliari_Sud/LConn2 -- _CN_255011550_380000_CN_255011551_380000/RConn2
  _CN_255011550_380000_CN_255011551_380000/RConn3 -- T_255011551_380000_Cagliari_Sud/LConn3 -- bus418/LConn1
  T_74210017__Pogliano/LConn1 -- Turbigo_Ospiate_CN_74210017_380000_CN_162828577_380000/RConn1
  T_74210017__Pogliano/LConn2 -- Turbigo_Ospiate_CN_74210017_380000_CN_162828577_380000/RConn2
  Turbigo_Ospiate_CN_74210017_380000_CN_162828577_380000/RConn3 -- T_74210017__Pogliano/LConn3 -- bus419/LConn1
  _CN_74943205_380000_CN_143585004_380000/RConn1 -- T_143585004_380000_San_Martino_in_XX/LConn1 -- Linea_352_CN_143585004_380000_CN_81931074_380000/RConn1
  _CN_74943205_380000_CN_143585004_380000/RConn2 -- T_143585004_380000_San_Martino_in_XX/LConn2 -- Linea_352_CN_143585004_380000_CN_81931074_380000/RConn2
  _CN_74943205_380000_CN_143585004_380000/RConn3 -- T_143585004_380000_San_Martino_in_XX/LConn3 -- Linea_352_CN_143585004_380000_CN_81931074_380000/RConn3 -- bus420/LConn1
  T_118987056_380000_Selargius/LConn1 -- Ittiri_Selargius_CN_144005863_380000_CN_118987056_380000/RConn1
  T_118987056_380000_Selargius/LConn2 -- Ittiri_Selargius_CN_144005863_380000_CN_118987056_380000/RConn2
  Ittiri_Selargius_CN_144005863_380000_CN_118987056_380000/RConn3 -- T_118987056_380000_Selargius/LConn3 -- bus421/LConn1
  T_96190189_380000_San_Giacomo_380/LConn1 -- Teramo_San_Giacomo_380_CN_96190189_380000_CN_61626687_380000/RConn1
  T_96190189_380000_San_Giacomo_380/LConn2 -- Teramo_San_Giacomo_380_CN_96190189_380000_CN_61626687_380000/RConn2
  Teramo_San_Giacomo_380_CN_96190189_380000_CN_61626687_380000/RConn3 -- T_96190189_380000_San_Giacomo_380/LConn3 -- bus422/LConn1
  T_98900549_380000_Ferrera_Erbognone/LConn1 -- _CN_98900549_380000_CN402288342/RConn1
  T_98900549_380000_Ferrera_Erbognone/LConn2 -- _CN_98900549_380000_CN402288342/RConn2
  _CN_98900549_380000_CN402288342/RConn3 -- T_98900549_380000_Ferrera_Erbognone/LConn3 -- bus423/LConn1
  Chiari_Travagliato_CN_120356593_380000_CN_72475426_380000/RConn1 -- T_72475426_380000_Chiari/LConn1 -- Chiari_Gorlago_CN_72475426_380000_CN_42206116_380000/LConn1
  Chiari_Travagliato_CN_120356593_380000_CN_72475426_380000/RConn2 -- T_72475426_380000_Chiari/LConn2 -- Chiari_Gorlago_CN_72475426_380000_CN_42206116_380000/LConn2
  Chiari_Travagliato_CN_120356593_380000_CN_72475426_380000/RConn3 -- T_72475426_380000_Chiari/LConn3 -- Chiari_Gorlago_CN_72475426_380000_CN_42206116_380000/LConn3 -- bus424/LConn1
  Santa_Lucia_Roma_Ovest_CN_82762493_380000_CN_80399102_380000/RConn1 -- T_80399102_380000_Roma_Ovest/LConn1 -- Roma_Sud_Roma_Ovest_CN_80399102_380000_CN_76705565_380000/RConn1
  Santa_Lucia_Roma_Ovest_CN_82762493_380000_CN_80399102_380000/RConn2 -- T_80399102_380000_Roma_Ovest/LConn2 -- Roma_Sud_Roma_Ovest_CN_80399102_380000_CN_76705565_380000/RConn2
  Santa_Lucia_Roma_Ovest_CN_82762493_380000_CN_80399102_380000/RConn3 -- T_80399102_380000_Roma_Ovest/LConn3 -- Roma_Sud_Roma_Ovest_CN_80399102_380000_CN_76705565_380000/RConn3 -- bus425/LConn1
  T_82767145_380000_Tirreno_Power_Torrevaldaliga/LConn1 -- _CN_82762493_380000_CN_82767145_380000/RConn1
  T_82767145_380000_Tirreno_Power_Torrevaldaliga/LConn2 -- _CN_82762493_380000_CN_82767145_380000/RConn2
  _CN_82762493_380000_CN_82767145_380000/RConn3 -- T_82767145_380000_Tirreno_Power_Torrevaldaliga/LConn3 -- bus426/LConn1
  T_145665799_380000_Brindisi_Nord_380/LConn1 -- _CN_145665799_380000_CN_60919237_380000/RConn1
  T_145665799_380000_Brindisi_Nord_380/LConn2 -- _CN_145665799_380000_CN_60919237_380000/RConn2
  _CN_145665799_380000_CN_60919237_380000/RConn3 -- T_145665799_380000_Brindisi_Nord_380/LConn3 -- bus427/LConn1
  "G_61814451_Centrale_termoelettrica_\"Federico_II\""/RConn1 -- _CN_60888331_380000_CN61814451/RConn1
  "G_61814451_Centrale_termoelettrica_\"Federico_II\""/RConn2 -- _CN_60888331_380000_CN61814451/RConn2
  _CN_60888331_380000_CN61814451/RConn3 -- "G_61814451_Centrale_termoelettrica_\"Federico_II\""/RConn3 -- bus428/LConn1
  Sparanise_Santa_Maria_Capua_Vetere_CN_93860115_380000_CN_132450233_380000/RConn1 -- T_132450233_380000_Sparanise/LConn1 -- Sparanise_Garigliano_CN_132450233_380000_CN_83872215_380000/RConn1 -- _CN_132450233_380000_CN132450235/LConn1
  Sparanise_Santa_Maria_Capua_Vetere_CN_93860115_380000_CN_132450233_380000/RConn2 -- T_132450233_380000_Sparanise/LConn2 -- Sparanise_Garigliano_CN_132450233_380000_CN_83872215_380000/RConn2 -- _CN_132450233_380000_CN132450235/LConn2
  Sparanise_Santa_Maria_Capua_Vetere_CN_93860115_380000_CN_132450233_380000/RConn3 -- T_132450233_380000_Sparanise/LConn3 -- Sparanise_Garigliano_CN_132450233_380000_CN_83872215_380000/RConn3 -- _CN_132450233_380000_CN132450235/LConn3 -- bus429/LConn1
  T_100407575_380000_Fusina_Termica_sezione_1_400/LConn1 -- _CN_100407575_380000_CN244931645/LConn1
  T_100407575_380000_Fusina_Termica_sezione_1_400/LConn2 -- _CN_100407575_380000_CN244931645/LConn2
  _CN_100407575_380000_CN244931645/LConn3 -- T_100407575_380000_Fusina_Termica_sezione_1_400/LConn3 -- bus430/LConn1
  _CN_100407575_380000_CN244931645/RConn1 -- "G_244931645_Centrale_termoelettrica_\"Andrea_Palladio\""/RConn1 -- _CN_59153311_380000_CN244931645/RConn1
  _CN_100407575_380000_CN244931645/RConn2 -- "G_244931645_Centrale_termoelettrica_\"Andrea_Palladio\""/RConn2 -- _CN_59153311_380000_CN244931645/RConn2
  _CN_100407575_380000_CN244931645/RConn3 -- "G_244931645_Centrale_termoelettrica_\"Andrea_Palladio\""/RConn3 -- _CN_59153311_380000_CN244931645/RConn3 -- bus431/LConn1
  Roma_Sud_Aprilia_380_CN_76705565_380000_CN_172302572_380000/RConn1 -- T_172302572_380000_Aprilia_380/LConn1 -- Latina_Aprilia_380_CN_339704025_380000_CN_172302572_380000/RConn1
  Roma_Sud_Aprilia_380_CN_76705565_380000_CN_172302572_380000/RConn2 -- T_172302572_380000_Aprilia_380/LConn2 -- Latina_Aprilia_380_CN_339704025_380000_CN_172302572_380000/RConn2
  Roma_Sud_Aprilia_380_CN_76705565_380000_CN_172302572_380000/RConn3 -- T_172302572_380000_Aprilia_380/LConn3 -- Latina_Aprilia_380_CN_339704025_380000_CN_172302572_380000/RConn3 -- bus432/LConn1
  Chiari_Gorlago_CN_72475426_380000_CN_42206116_380000/RConn1 -- T_42206116_380000_Gorlago/LConn1 -- _CN_72466334_380000_CN_42206116_380000/RConn1
  Chiari_Gorlago_CN_72475426_380000_CN_42206116_380000/RConn2 -- T_42206116_380000_Gorlago/LConn2 -- _CN_72466334_380000_CN_42206116_380000/RConn2
  Chiari_Gorlago_CN_72475426_380000_CN_42206116_380000/RConn3 -- T_42206116_380000_Gorlago/LConn3 -- _CN_72466334_380000_CN_42206116_380000/RConn3 -- bus433/LConn1
  _CN_68299044_380000_CN_162960205_380000/RConn1 -- T_68299044_380000_Brugherio___Smistamento_elettrico_TERNA/LConn1 -- Bovisio_Brugherio_CN_68299044_380000_CN_74677138_380000/RConn1
  _CN_68299044_380000_CN_162960205_380000/RConn2 -- T_68299044_380000_Brugherio___Smistamento_elettrico_TERNA/LConn2 -- Bovisio_Brugherio_CN_68299044_380000_CN_74677138_380000/RConn2
  _CN_68299044_380000_CN_162960205_380000/RConn3 -- T_68299044_380000_Brugherio___Smistamento_elettrico_TERNA/LConn3 -- Bovisio_Brugherio_CN_68299044_380000_CN_74677138_380000/RConn3 -- bus434/LConn1
  _CN_145665323_380000_CN_60919237_380000/RConn1 -- T_145665323__/LConn1 -- _CN_145665323_380000_CN_145665862_380000/LConn1
  _CN_145665323_380000_CN_60919237_380000/RConn2 -- T_145665323__/LConn2 -- _CN_145665323_380000_CN_145665862_380000/LConn2
  _CN_145665323_380000_CN_60919237_380000/RConn3 -- T_145665323__/LConn3 -- _CN_145665323_380000_CN_145665862_380000/LConn3 -- bus435/LConn1
  T_145665862_380000_Enipower_Brindisi_380/LConn1 -- _CN_145665323_380000_CN_145665862_380000/RConn1
  T_145665862_380000_Enipower_Brindisi_380/LConn2 -- _CN_145665323_380000_CN_145665862_380000/RConn2
  _CN_145665323_380000_CN_145665862_380000/RConn3 -- T_145665862_380000_Enipower_Brindisi_380/LConn3 -- bus436/LConn1
  G_61012012_Centrale_Idroelettrica_di_Ceprano/RConn1 -- Latina_Ceprano_CN_339704025_380000_CN61012012/RConn1
  G_61012012_Centrale_Idroelettrica_di_Ceprano/RConn2 -- Latina_Ceprano_CN_339704025_380000_CN61012012/RConn2
  Latina_Ceprano_CN_339704025_380000_CN61012012/RConn3 -- G_61012012_Centrale_Idroelettrica_di_Ceprano/RConn3 -- bus437/LConn1
  Casanova___Magliano_CN_99694910_380000_CN_99826025_380000/RConn1 -- T_99826025_380000_Casanova/LConn1 -- Piossasco_Casanova_CN_99826025_380000_CN_98902899_380000/LConn1 -- Casanova_Chivasso_Termica_CN_105581403_380000_CN_99826025_380000/LConn1
  Casanova___Magliano_CN_99694910_380000_CN_99826025_380000/RConn2 -- T_99826025_380000_Casanova/LConn2 -- Piossasco_Casanova_CN_99826025_380000_CN_98902899_380000/LConn2 -- Casanova_Chivasso_Termica_CN_105581403_380000_CN_99826025_380000/LConn2
  Casanova___Magliano_CN_99694910_380000_CN_99826025_380000/RConn3 -- T_99826025_380000_Casanova/LConn3 -- Piossasco_Casanova_CN_99826025_380000_CN_98902899_380000/LConn3 -- bus438/LConn1 -- Casanova_Chivasso_Termica_CN_105581403_380000_CN_99826025_380000/LConn3
  Magliano_Piossasco_CN_99694910_380000_CN_98902899_380000/RConn1 -- T_98902899_380000_Piossasco/LConn1 -- Piossasco_Casanova_CN_99826025_380000_CN_98902899_380000/RConn1 -- _CN_98902899_380000_CN401799924/LConn1 -- Piossasco___Leinì_CN_98902899_380000_CN_105153431_380000/LConn1
  Magliano_Piossasco_CN_99694910_380000_CN_98902899_380000/RConn2 -- T_98902899_380000_Piossasco/LConn2 -- Piossasco_Casanova_CN_99826025_380000_CN_98902899_380000/RConn2 -- _CN_98902899_380000_CN401799924/LConn2 -- Piossasco___Leinì_CN_98902899_380000_CN_105153431_380000/LConn2
  Magliano_Piossasco_CN_99694910_380000_CN_98902899_380000/RConn3 -- T_98902899_380000_Piossasco/LConn3 -- Piossasco_Casanova_CN_99826025_380000_CN_98902899_380000/RConn3 -- _CN_98902899_380000_CN401799924/LConn3 -- Piossasco___Leinì_CN_98902899_380000_CN_105153431_380000/LConn3 -- bus439/LConn1
  T_414663585_380000_Rosen/LConn1 -- _CN_116240715_380000_CN_414663585_380000/RConn1
  T_414663585_380000_Rosen/LConn2 -- _CN_116240715_380000_CN_414663585_380000/RConn2
  _CN_116240715_380000_CN_414663585_380000/RConn3 -- T_414663585_380000_Rosen/LConn3 -- bus440/LConn1
  Turano_Tavazzano_CN_162960205_380000_CN_339104227_380000/RConn1 -- T_339104227_380000_Turano_centrale/LConn1 -- San_Rocco_Turano_CN_339104227_380000_CN_93315059_380000/RConn1
  Turano_Tavazzano_CN_162960205_380000_CN_339104227_380000/RConn2 -- T_339104227_380000_Turano_centrale/LConn2 -- San_Rocco_Turano_CN_339104227_380000_CN_93315059_380000/RConn2
  Turano_Tavazzano_CN_162960205_380000_CN_339104227_380000/RConn3 -- T_339104227_380000_Turano_centrale/LConn3 -- San_Rocco_Turano_CN_339104227_380000_CN_93315059_380000/RConn3 -- bus441/LConn1
  T_284418385_380000_Stazione_Elettrica_Villafranca_2/LConn1 -- _CN_284418385_380000_CN_110660048_380000/LConn1
  T_284418385_380000_Stazione_Elettrica_Villafranca_2/LConn2 -- _CN_284418385_380000_CN_110660048_380000/LConn2
  _CN_284418385_380000_CN_110660048_380000/LConn3 -- T_284418385_380000_Stazione_Elettrica_Villafranca_2/LConn3 -- bus442/LConn1
  T_110660048__/LConn1 -- _CN_284418385_380000_CN_110660048_380000/RConn1
  T_110660048__/LConn2 -- _CN_284418385_380000_CN_110660048_380000/RConn2
  _CN_284418385_380000_CN_110660048_380000/RConn3 -- T_110660048__/LConn3 -- bus443/LConn1
  Casanova_Chivasso_Termica_CN_105581403_380000_CN_99826025_380000/RConn1 -- T_105581403_380000_Chivasso_Termica_380kV/LConn1 -- Chivasso_Termica___Rondissone_CN_105581403_380000_CN_74869121_380000/RConn1
  Casanova_Chivasso_Termica_CN_105581403_380000_CN_99826025_380000/RConn2 -- T_105581403_380000_Chivasso_Termica_380kV/LConn2 -- Chivasso_Termica___Rondissone_CN_105581403_380000_CN_74869121_380000/RConn2
  Casanova_Chivasso_Termica_CN_105581403_380000_CN_99826025_380000/RConn3 -- T_105581403_380000_Chivasso_Termica_380kV/LConn3 -- Chivasso_Termica___Rondissone_CN_105581403_380000_CN_74869121_380000/RConn3 -- bus444/LConn1
  Paternò_Chiaramonte_Gulfi_CN_57384507_380000_CN_61157826_380000/RConn1 -- T_61157826_380000_Barca___Paternò/LConn1 -- Elettrodotto_Sorgente___Paternò_CN_110138220_380000_CN_61157826_380000/RConn1
  Paternò_Chiaramonte_Gulfi_CN_57384507_380000_CN_61157826_380000/RConn2 -- T_61157826_380000_Barca___Paternò/LConn2 -- Elettrodotto_Sorgente___Paternò_CN_110138220_380000_CN_61157826_380000/RConn2
  Paternò_Chiaramonte_Gulfi_CN_57384507_380000_CN_61157826_380000/RConn3 -- T_61157826_380000_Barca___Paternò/LConn3 -- Elettrodotto_Sorgente___Paternò_CN_110138220_380000_CN_61157826_380000/RConn3 -- bus445/LConn1
  T_339706878_380000_Ceprano/LConn1 -- Garigliano_Ceprano_CN_339706878_380000_CN_83872215_380000/RConn1
  T_339706878_380000_Ceprano/LConn2 -- Garigliano_Ceprano_CN_339706878_380000_CN_83872215_380000/RConn2
  Garigliano_Ceprano_CN_339706878_380000_CN_83872215_380000/RConn3 -- T_339706878_380000_Ceprano/LConn3 -- bus446/LConn1
  G_401799924_Centrale_Idroelettrica_Enel/RConn1 -- _CN_98902899_380000_CN401799924/RConn1
  G_401799924_Centrale_Idroelettrica_Enel/RConn2 -- _CN_98902899_380000_CN401799924/RConn2
  _CN_98902899_380000_CN401799924/RConn3 -- G_401799924_Centrale_Idroelettrica_Enel/RConn3 -- bus447/LConn1
  Piossasco___Leinì_CN_98902899_380000_CN_105153431_380000/RConn1 -- T_105153431_380000_Leinì/LConn1 -- Rondissone_Leini_CN_74869121_380000_CN_105153431_380000/RConn1 -- _CN_105153431_380000_CN_332123608_380000/LConn1
  Piossasco___Leinì_CN_98902899_380000_CN_105153431_380000/RConn2 -- T_105153431_380000_Leinì/LConn2 -- Rondissone_Leini_CN_74869121_380000_CN_105153431_380000/RConn2 -- _CN_105153431_380000_CN_332123608_380000/LConn2
  Piossasco___Leinì_CN_98902899_380000_CN_105153431_380000/RConn3 -- T_105153431_380000_Leinì/LConn3 -- Rondissone_Leini_CN_74869121_380000_CN_105153431_380000/RConn3 -- _CN_105153431_380000_CN_332123608_380000/LConn3 -- bus448/LConn1
  G_81944353_Centrale_termoelettrica_di_Porto_Tolle/RConn1 -- _CN_81929591_380000_CN81944353/RConn1
  G_81944353_Centrale_termoelettrica_di_Porto_Tolle/RConn2 -- _CN_81929591_380000_CN81944353/RConn2
  _CN_81929591_380000_CN81944353/RConn3 -- G_81944353_Centrale_termoelettrica_di_Porto_Tolle/RConn3 -- bus449/LConn1
  T_155158689_380000_Adria_Sud/LConn1 -- _CN_81929591_380000_CN_155158689_380000/RConn1
  T_155158689_380000_Adria_Sud/LConn2 -- _CN_81929591_380000_CN_155158689_380000/RConn2
  _CN_81929591_380000_CN_155158689_380000/RConn3 -- T_155158689_380000_Adria_Sud/LConn3 -- bus450/LConn1
  T_421827451_380000_La_Casella_centrale/LConn1 -- _CN_421827451_380000_CN_107438024_380000/LConn1
  T_421827451_380000_La_Casella_centrale/LConn2 -- _CN_421827451_380000_CN_107438024_380000/LConn2
  _CN_421827451_380000_CN_107438024_380000/LConn3 -- T_421827451_380000_La_Casella_centrale/LConn3 -- bus451/LConn1
  _CN_421827451_380000_CN_107438024_380000/RConn1 -- T_107438024_380000_La_Casella/LConn1 -- _CN_107438024_380000_CN_202271565_380000/RConn1
  _CN_421827451_380000_CN_107438024_380000/RConn2 -- T_107438024_380000_La_Casella/LConn2 -- _CN_107438024_380000_CN_202271565_380000/RConn2
  _CN_421827451_380000_CN_107438024_380000/RConn3 -- T_107438024_380000_La_Casella/LConn3 -- _CN_107438024_380000_CN_202271565_380000/RConn3 -- bus452/LConn1
  T_421827453_380000_Piacenza/LConn1 -- Piacenza_San_Rocco_CN_421827453_380000_CN_93315059_380000/RConn1
  T_421827453_380000_Piacenza/LConn2 -- Piacenza_San_Rocco_CN_421827453_380000_CN_93315059_380000/RConn2
  Piacenza_San_Rocco_CN_421827453_380000_CN_93315059_380000/RConn3 -- T_421827453_380000_Piacenza/LConn3 -- bus453/LConn1
  G_161471016_/RConn1 -- _CN_59219335_380000_CN161471016/RConn1
  G_161471016_/RConn2 -- _CN_59219335_380000_CN161471016/RConn2
  _CN_59219335_380000_CN161471016/RConn3 -- G_161471016_/RConn3 -- bus454/LConn1
  G_259565911_Centrale_di_Bargi/RConn1 -- _CN_114931087_380000_CN259565911/RConn1
  G_259565911_Centrale_di_Bargi/RConn2 -- _CN_114931087_380000_CN259565911/RConn2
  _CN_114931087_380000_CN259565911/RConn3 -- G_259565911_Centrale_di_Bargi/RConn3 -- bus455/LConn1
  T_332123608__/LConn1 -- _CN_105153431_380000_CN_332123608_380000/RConn1
  T_332123608__/LConn2 -- _CN_105153431_380000_CN_332123608_380000/RConn2
  _CN_105153431_380000_CN_332123608_380000/RConn3 -- T_332123608__/LConn3 -- bus456/LConn1
  T_75602396_380000_Pian_Camuno/LConn1 -- _CN_72466334_380000_CN_75602396_380000/RConn1
  T_75602396_380000_Pian_Camuno/LConn2 -- _CN_72466334_380000_CN_75602396_380000/RConn2
  _CN_72466334_380000_CN_75602396_380000/RConn3 -- T_75602396_380000_Pian_Camuno/LConn3 -- bus457/LConn1
  G_132450235_/RConn1 -- _CN_132450233_380000_CN132450235/RConn1
  G_132450235_/RConn2 -- _CN_132450233_380000_CN132450235/RConn2
  _CN_132450233_380000_CN132450235/RConn3 -- G_132450235_/RConn3 -- bus458/LConn1
  T_116519166_380000_Isp_Cremona/LConn1 -- _CN_116518388_380000_CN_116519166_380000/RConn1
  T_116519166_380000_Isp_Cremona/LConn2 -- _CN_116518388_380000_CN_116519166_380000/RConn2
  _CN_116518388_380000_CN_116519166_380000/RConn3 -- T_116519166_380000_Isp_Cremona/LConn3 -- bus459/LConn1
  T_152457216_220000_San_Pancrazio/RConn1 -- L_152457216/LConn1
  T_152457216_220000_San_Pancrazio/RConn2 -- L_152457216/LConn2
  L_152457216/LConn3 -- T_152457216_220000_San_Pancrazio/RConn3 -- bus460/LConn1
  T_42862642_220000_Lana/RConn1 -- L_42862642/LConn1
  T_42862642_220000_Lana/RConn2 -- L_42862642/LConn2
  L_42862642/LConn3 -- T_42862642_220000_Lana/RConn3 -- bus461/LConn1
  T_153548074_220000_Castelbello/RConn1 -- L_153548074/LConn1
  T_153548074_220000_Castelbello/RConn2 -- L_153548074/LConn2
  L_153548074/LConn3 -- T_153548074_220000_Castelbello/RConn3 -- bus462/LConn1
  T_96727258_220000_Eppan___Appiano/RConn1 -- L_96727258/LConn1
  T_96727258_220000_Eppan___Appiano/RConn2 -- L_96727258/LConn2
  L_96727258/LConn3 -- T_96727258_220000_Eppan___Appiano/RConn3 -- bus463/LConn1
  T_205597560_220000_/RConn1 -- L_205597560/LConn1
  T_205597560_220000_/RConn2 -- L_205597560/LConn2
  L_205597560/LConn3 -- T_205597560_220000_/RConn3 -- bus464/LConn1
  T_102675884_220000_Avise/RConn1 -- L_102675884/LConn1
  T_102675884_220000_Avise/RConn2 -- L_102675884/LConn2
  L_102675884/LConn3 -- T_102675884_220000_Avise/RConn3 -- bus465/LConn1
  T_102185362_220000_Villeneuve/RConn1 -- L_102185362/LConn1
  T_102185362_220000_Villeneuve/RConn2 -- L_102185362/LConn2
  L_102185362/LConn3 -- T_102185362_220000_Villeneuve/RConn3 -- bus466/LConn1
  T_103127416_220000_Valpelline_G1/RConn1 -- L_103127416/LConn1
  T_103127416_220000_Valpelline_G1/RConn2 -- L_103127416/LConn2
  L_103127416/LConn3 -- T_103127416_220000_Valpelline_G1/RConn3 -- bus467/LConn1
  T_132723724__/RConn1 -- L_132723724/LConn1
  T_132723724__/RConn2 -- L_132723724/LConn2
  L_132723724/LConn3 -- T_132723724__/RConn3 -- bus468/LConn1
  T_376502663_220000_Colli_Aminei/RConn1 -- L_376502663/LConn1
  T_376502663_220000_Colli_Aminei/RConn2 -- L_376502663/LConn2
  L_376502663/LConn3 -- T_376502663_220000_Colli_Aminei/RConn3 -- bus469/LConn1
  T_114661587_380000_Patria/RConn1 -- L_114661587/LConn1
  T_114661587_380000_Patria/RConn2 -- L_114661587/LConn2
  L_114661587/LConn3 -- T_114661587_380000_Patria/RConn3 -- bus470/LConn1
  T_202178573_220000_Ercolano/RConn1 -- L_202178573/LConn1
  T_202178573_220000_Ercolano/RConn2 -- L_202178573/LConn2
  L_202178573/LConn3 -- T_202178573_220000_Ercolano/RConn3 -- bus471/LConn1
  T_132645607_220000_Torre_Nord/RConn1 -- L_132645607/LConn1
  T_132645607_220000_Torre_Nord/RConn2 -- L_132645607/LConn2
  L_132645607/LConn3 -- T_132645607_220000_Torre_Nord/RConn3 -- bus472/LConn1
  T_132643428_220000_San_Valentino/RConn1 -- L_132643428/LConn1
  T_132643428_220000_San_Valentino/RConn2 -- L_132643428/LConn2
  L_132643428/LConn3 -- T_132643428_220000_San_Valentino/RConn3 -- bus473/LConn1
  T_202179060_220000_San_Sebastiano/RConn1 -- L_202179060/LConn1
  T_202179060_220000_San_Sebastiano/RConn2 -- L_202179060/LConn2
  L_202179060/LConn3 -- T_202179060_220000_San_Sebastiano/RConn3 -- bus474/LConn1
  T_338969614_220000;150000_San_Filippo_del_Mela_gruppi_1,2,3,4/RConn1 -- L_338969614/LConn1
  T_338969614_220000;150000_San_Filippo_del_Mela_gruppi_1,2,3,4/RConn2 -- L_338969614/LConn2
  L_338969614/LConn3 -- T_338969614_220000;150000_San_Filippo_del_Mela_gruppi_1,2,3,4/RConn3 -- bus475/LConn1
  T_98427407_220000_Trino_220_kV/RConn1 -- L_98427407/LConn1
  T_98427407_220000_Trino_220_kV/RConn2 -- L_98427407/LConn2
  L_98427407/LConn3 -- T_98427407_220000_Trino_220_kV/RConn3 -- bus476/LConn1
  T_335012182_220000_Balzola_Stazione/RConn1 -- L_335012182/LConn1
  T_335012182_220000_Balzola_Stazione/RConn2 -- L_335012182/LConn2
  L_335012182/LConn3 -- T_335012182_220000_Balzola_Stazione/RConn3 -- bus477/LConn1
  T_98638424_220000_Vercelli_Nord/RConn1 -- L_98638424/LConn1
  T_98638424_220000_Vercelli_Nord/RConn2 -- L_98638424/LConn2
  L_98638424/LConn3 -- T_98638424_220000_Vercelli_Nord/RConn3 -- bus478/LConn1
  T_105462289_220000_Ponte/RConn1 -- L_105462289/LConn1
  T_105462289_220000_Ponte/RConn2 -- L_105462289/LConn2
  L_105462289/LConn3 -- T_105462289_220000_Ponte/RConn3 -- bus479/LConn1
  T_103418587_220000_Verampio/RConn1 -- L_103418587/LConn1
  T_103418587_220000_Verampio/RConn2 -- L_103418587/LConn2
  L_103418587/LConn3 -- T_103418587_220000_Verampio/RConn3 -- bus480/LConn1
  T_50589203_220000_Misterbianco/RConn1 -- L_50589203/LConn1
  T_50589203_220000_Misterbianco/RConn2 -- L_50589203/LConn2
  L_50589203/LConn3 -- T_50589203_220000_Misterbianco/RConn3 -- bus481/LConn1
  T_110138220_380000_Sorgente/RConn1 -- L_110138220/LConn1
  T_110138220_380000_Sorgente/RConn2 -- L_110138220/LConn2
  L_110138220/LConn3 -- T_110138220_380000_Sorgente/RConn3 -- bus482/LConn1
  T_376642649_220000_Torretta/RConn1 -- L_376642649/LConn1
  T_376642649_220000_Torretta/RConn2 -- L_376642649/LConn2
  L_376642649/LConn3 -- T_376642649_220000_Torretta/RConn3 -- bus483/LConn1
  T_79879307_220000_Sesto_San_Giovanni/RConn1 -- L_79879307/LConn1
  T_79879307_220000_Sesto_San_Giovanni/RConn2 -- L_79879307/LConn2
  L_79879307/LConn3 -- T_79879307_220000_Sesto_San_Giovanni/RConn3 -- bus484/LConn1
  T_141046481_220000_Sottostazione_elettrica_Oristano/RConn1 -- L_141046481/LConn1
  T_141046481_220000_Sottostazione_elettrica_Oristano/RConn2 -- L_141046481/LConn2
  L_141046481/LConn3 -- T_141046481_220000_Sottostazione_elettrica_Oristano/RConn3 -- bus485/LConn1
  T_408799290_220000_Sulcis_Centrale/RConn1 -- L_408799290/LConn1
  T_408799290_220000_Sulcis_Centrale/RConn2 -- L_408799290/LConn2
  L_408799290/LConn3 -- T_408799290_220000_Sulcis_Centrale/RConn3 -- bus486/LConn1
  T_61743815_380000;220000;150000_Codrongianos/RConn4 -- L_61743815/LConn1
  T_61743815_380000;220000;150000_Codrongianos/RConn5 -- L_61743815/LConn2
  L_61743815/LConn3 -- T_61743815_380000;220000;150000_Codrongianos/RConn6 -- bus487/LConn1
  T_103381531_380000_Taranto_Nord/RConn1 -- L_103381531/LConn1
  T_103381531_380000_Taranto_Nord/RConn2 -- L_103381531/LConn2
  L_103381531/LConn3 -- T_103381531_380000_Taranto_Nord/RConn3 -- bus488/LConn1
  T_377300897_220000_Villa_Castelli/RConn1 -- L_377300897/LConn1
  T_377300897_220000_Villa_Castelli/RConn2 -- L_377300897/LConn2
  L_377300897/LConn3 -- T_377300897_220000_Villa_Castelli/RConn3 -- bus489/LConn1
  T_185576620_220000_/RConn1 -- L_185576620/LConn1
  T_185576620_220000_/RConn2 -- L_185576620/LConn2
  L_185576620/LConn3 -- T_185576620_220000_/RConn3 -- bus490/LConn1
  T_104321356_220000_Pisticci/RConn1 -- L_104321356/LConn1
  T_104321356_220000_Pisticci/RConn2 -- L_104321356/LConn2
  L_104321356/LConn3 -- T_104321356_220000_Pisticci/RConn3 -- bus491/LConn1
  T_185425637__/RConn1 -- L_185425637/LConn1
  T_185425637__/RConn2 -- L_185425637/LConn2
  L_185425637/LConn3 -- T_185425637__/RConn3 -- bus492/LConn1
  T_377830944_220000_Torino_Nord/RConn1 -- L_377830944/LConn1
  T_377830944_220000_Torino_Nord/RConn2 -- L_377830944/LConn2
  L_377830944/LConn3 -- T_377830944_220000_Torino_Nord/RConn3 -- bus493/LConn1
  T_332123606__/RConn1 -- L_332123606/LConn1
  T_332123606__/RConn2 -- L_332123606/LConn2
  L_332123606/LConn3 -- T_332123606__/RConn3 -- bus494/LConn1
  T_332123607__/RConn1 -- L_332123607/LConn1
  T_332123607__/RConn2 -- L_332123607/LConn2
  L_332123607/LConn3 -- T_332123607__/RConn3 -- bus495/LConn1
  T_187150881_220000_Mucone_primo_salto/RConn1 -- L_187150881/LConn1
  T_187150881_220000_Mucone_primo_salto/RConn2 -- L_187150881/LConn2
  L_187150881/LConn3 -- T_187150881_220000_Mucone_primo_salto/RConn3 -- bus496/LConn1
  T_187149304_220000_Terranova/RConn1 -- L_187149304/LConn1
  T_187149304_220000_Terranova/RConn2 -- L_187149304/LConn2
  L_187149304/LConn3 -- T_187149304_220000_Terranova/RConn3 -- bus497/LConn1
  T_103974946_220000_Teksid_Carmagnola/RConn1 -- L_103974946/LConn1
  T_103974946_220000_Teksid_Carmagnola/RConn2 -- L_103974946/LConn2
  L_103974946/LConn3 -- T_103974946_220000_Teksid_Carmagnola/RConn3 -- bus498/LConn1
  T_99826025_380000_Casanova/RConn1 -- L_99826025/LConn1
  T_99826025_380000_Casanova/RConn2 -- L_99826025/LConn2
  L_99826025/LConn3 -- T_99826025_380000_Casanova/RConn3 -- bus499/LConn1
  T_104239286_220000_Bistagno/RConn1 -- L_104239286/LConn1
  T_104239286_220000_Bistagno/RConn2 -- L_104239286/LConn2
  L_104239286/LConn3 -- T_104239286_220000_Bistagno/RConn3 -- bus500/LConn1
  T_103525675_220000_Moncalieri_AEM/RConn1 -- L_103525675/LConn1
  T_103525675_220000_Moncalieri_AEM/RConn2 -- L_103525675/LConn2
  L_103525675/LConn3 -- T_103525675_220000_Moncalieri_AEM/RConn3 -- bus501/LConn1
  T_108050523_220000;132000_FS_Nomentana/RConn1 -- L_108050523/LConn1
  T_108050523_220000;132000_FS_Nomentana/RConn2 -- L_108050523/LConn2
  L_108050523/LConn3 -- T_108050523_220000;132000_FS_Nomentana/RConn3 -- bus502/LConn1
  T_80517630_380000_Roma_Nord_smistamento_energia_elettrica_TERNA/RConn1 -- L_80517630/LConn1
  T_80517630_380000_Roma_Nord_smistamento_energia_elettrica_TERNA/RConn2 -- L_80517630/LConn2
  L_80517630/LConn3 -- T_80517630_380000_Roma_Nord_smistamento_energia_elettrica_TERNA/RConn3 -- bus503/LConn1
